simulink model "deltino"  (R2021b)
settings: Solver=VariableStepAuto  StartTime=0.0  StopTime=inf  FixedStep=0.0001  RelTol=1e-3
values from neighbouring files (symbols this model uses):
  alpha1 = 0    [compute_deltino_dyn_parallel.m]
  alpha2 = 2/3*pi    (= 2.09439510239)    [compute_deltino_dyn_parallel.m]
  alpha3 = 4/3*pi    (= 4.18879020479)    [compute_deltino_dyn_parallel.m]
  H = 0.05    [main.m]
  J_T = [J_1', J_2', J_3', J_4']    [main.m]
  K_d = 10    [main.m]
  K_el = 10000    [main.m]
  K_i = 1    [main.m]
  K_p = 200    [main.m]
  K_v = 10    [main.m]
  mu = 0.8    [main.m]
  ni_0 = zeros(18,1)    [main.m]
  offset1 = [l1/2; l2/2; -h/2]    [compute_deltino_dyn_parallel.m]    (also in main.m = [+l1/2; +l2/2; -h/2])
  offset2 = [l1/2; -l2/2; -h/2]    [compute_deltino_dyn_parallel.m]    (also in main.m = [+l1/2; -l2/2; -h/2])
  offset3 = [-l1/2; -l2/2; -h/2]    [compute_deltino_dyn_parallel.m]    (also in main.m)
  offset4 = [-l1/2; l2/2; -h/2]    [compute_deltino_dyn_parallel.m]    (also in main.m = [-l1/2; +l2/2; -h/2])
  p_leg1_0 = forward_kin(theta_leg1_0)    [main.m]
  p_leg2_0 = forward_kin(theta_leg2_0)    [main.m]
  p_leg3_0 = forward_kin(theta_leg3_0)    [main.m]
  p_leg4_0 = forward_kin(theta_leg4_0)    [main.m]
  points_ccw = [+0.1,  0.00 ... (first row only)    [main.m]
  points_cw = [-0.1,  0.00 ... (first row only)    [main.m]
  q_0 = [base_0; ypr_0; theta_leg1_0; ee_leg1_0; theta_leg2_0; ee_leg2_0;        theta_leg3_0; ee_leg3_0; theta_leg4_0; ee_leg4_0;]    [main.m]
  ratio = 2    [main.m]
  steps = 4+2*ratio    (= 8)    [main.m]
  theta_leg1_0 = [pi/6; pi/6; pi/6]    [main.m]
  theta_leg2_0 = [pi/6; pi/6; pi/6]    [main.m]
  theta_leg3_0 = [pi/6; pi/6; pi/6]    [main.m]
  theta_leg4_0 = [pi/6; pi/6; pi/6]    [main.m]
  ts = T/steps    (= 0.1875)    [main.m]
  ts2 = 3*ts    (= 0.5625)    [main.m]
  vel = 0.2    [main.m]
undefined symbols (not defined in the file or in its folder): l1, l_A, l_B, R, radius0, radius1, radius2, theta, WPs
libraries: simulink x14, dspsigops x12
(part 6 of 10)

== matlab function deltino/DELTINO DYNAMICS /compute_M ==
  data: q input; M output
function M = M(q)
%#codegen

%    This function was generated by the Symbolic Math Toolbox version 9.0.
%    03-May-2022 23:36:54
phi = q(4); zeta = q(5); psi = q(6);
th11 = q(7); th12 = q(8); th13 = q(9);
th21 = q(13); th22 = q(14); th23 = q(15);
th31 = q(19); th32 = q(20); th33 = q(21);
th41 = q(25); th42 = q(26); th43 = q(27);


t2 = cos(phi);
t3 = cos(psi);
t4 = cos(th11);
t5 = cos(th12);
t6 = cos(th13);
t7 = cos(th21);
t8 = cos(th22);
t9 = cos(th23);
t10 = cos(th31);
t11 = cos(th32);
t12 = cos(th33);
t13 = cos(th41);
t14 = cos(th42);
t15 = cos(th43);
t16 = cos(zeta);
t17 = sin(phi);
t18 = sin(psi);
t19 = sin(th11);
t20 = sin(th12);
t21 = sin(th13);
t22 = sin(th21);
t23 = sin(th22);
t24 = sin(th23);
t25 = sin(th31);
t26 = sin(th32);
t27 = sin(th33);
t28 = sin(th41);
t29 = sin(th42);
t30 = sin(th43);
t31 = sin(zeta);
t32 = psi.*2.0;
t33 = th11.*2.0;
t34 = th12.*2.0;
t35 = th13.*2.0;
t36 = th21.*2.0;
t37 = th22.*2.0;
t38 = th23.*2.0;
t39 = th31.*2.0;
t40 = th32.*2.0;
t41 = th33.*2.0;
t42 = th41.*2.0;
t43 = th42.*2.0;
t44 = th43.*2.0;
t94 = sqrt(3.0);
t95 = psi./2.0;
t96 = th12./2.0;
t97 = th13./2.0;
t98 = th22./2.0;
t99 = th23./2.0;
t100 = th32./2.0;
t101 = th33./2.0;
t102 = th42./2.0;
t103 = th43./2.0;
t45 = cos(t32);
t46 = t3.^2;
t47 = cos(t34);
t48 = cos(t35);
t49 = cos(t37);
t50 = cos(t38);
t51 = cos(t40);
t52 = cos(t41);
t53 = cos(t43);
t54 = cos(t44);
t55 = t4.^2;
t56 = t5.^2;
t57 = t6.^2;
t58 = t7.^2;
t59 = t8.^2;
t60 = t9.^2;
t61 = t10.^2;
t62 = t11.^2;
t63 = t12.^2;
t64 = t13.^2;
t65 = t14.^2;
t66 = t15.^2;
t67 = t16.^2;
t68 = sin(t32);
t69 = sin(t33);
t70 = sin(t34);
t71 = sin(t35);
t72 = sin(t36);
t73 = sin(t37);
t74 = sin(t38);
t75 = sin(t39);
t76 = sin(t40);
t77 = sin(t41);
t78 = sin(t42);
t79 = sin(t43);
t80 = sin(t44);
t81 = t2.*t3;
t82 = t2.*t18;
t83 = t3.*t17;
t84 = t5.*t31;
t85 = t6.*t31;
t86 = t8.*t31;
t87 = t9.*t31;
t88 = t11.*t31;
t89 = t12.*t31;
t90 = t14.*t31;
t91 = t15.*t31;
t92 = t17.*t18;
t93 = t18.*1.6e+1;
t104 = t4.*t31.*2.0;
t105 = t7.*t31.*2.0;
t106 = t10.*t31.*2.0;
t107 = t13.*t31.*2.0;
t108 = t18.*t19.*2.0;
t109 = t18.*t20.*2.0;
t110 = t18.*t21.*2.0;
t111 = t18.*t22.*2.0;
t112 = t18.*t23.*2.0;
t113 = t18.*t24.*2.0;
t114 = t18.*t25.*2.0;
t115 = t18.*t26.*2.0;
t116 = t18.*t27.*2.0;
t117 = t18.*t28.*2.0;
t118 = t18.*t29.*2.0;
t119 = t18.*t30.*2.0;
t120 = cos(t95);
t121 = cos(t96);
t122 = cos(t97);
t123 = cos(t98);
t124 = cos(t99);
t125 = cos(t100);
t126 = cos(t101);
t127 = cos(t102);
t128 = cos(t103);
t129 = t16./2.0;
t130 = sin(t95);
t131 = sin(t96);
t132 = sin(t97);
t133 = sin(t98);
t134 = sin(t99);
t135 = sin(t100);
t136 = sin(t101);
t137 = sin(t102);
t138 = sin(t103);
t139 = t31./2.0;
t142 = t3.*t16.*1.6e+1;
t152 = t4.*(3.0./2.0e+1);
t153 = t5.*(3.0./2.0e+1);
t154 = t6.*(3.0./2.0e+1);
t155 = t7.*(3.0./2.0e+1);
t156 = t8.*(3.0./2.0e+1);
t157 = t9.*(3.0./2.0e+1);
t158 = t10.*(3.0./2.0e+1);
t159 = t11.*(3.0./2.0e+1);
t160 = t12.*(3.0./2.0e+1);
t161 = t13.*(3.0./2.0e+1);
t162 = t14.*(3.0./2.0e+1);
t163 = t15.*(3.0./2.0e+1);
t164 = t16.*(6.0./2.5e+1);
t169 = t3.*(4.0./3.75e+2);
t180 = t3.*t16.*t19.*2.0;
t181 = t3.*t16.*t20.*2.0;
t182 = t3.*t16.*t21.*2.0;
t183 = t3.*t16.*t22.*2.0;
t184 = t3.*t16.*t23.*2.0;
t185 = t3.*t16.*t24.*2.0;
t186 = t3.*t16.*t25.*2.0;
t187 = t3.*t16.*t26.*2.0;
t188 = t3.*t16.*t27.*2.0;
t189 = t3.*t16.*t28.*2.0;
t190 = t3.*t16.*t29.*2.0;
t191 = t3.*t16.*t30.*2.0;
t195 = t2.*t16.*(7.0./2.0e+1);
t196 = t4.*t16.*(3.0./5.0e+1);
t197 = t7.*t16.*(3.0./5.0e+1);
t198 = t10.*t16.*(3.0./5.0e+1);
t199 = t13.*t16.*(3.0./5.0e+1);
t202 = t16.*t17.*(7.0./2.0e+1);
t204 = t19.*t31.*(3.0./5.0e+1);
t205 = t22.*t31.*(3.0./5.0e+1);
t206 = t25.*t31.*(3.0./5.0e+1);
t207 = t28.*t31.*(3.0./5.0e+1);
t209 = t3.*t4.*(3.0./1.0e+2);
t210 = t3.*t7.*(3.0./1.0e+2);
t211 = t3.*t10.*(3.0./2.5e+2);
t212 = t3.*t13.*(3.0./2.5e+2);
t222 = t3.*t19.*(3.0./5.0e+2);
t223 = t4.*t18.*(3.0./5.0e+2);
t224 = t3.*t22.*(3.0./5.0e+2);
t225 = t7.*t18.*(3.0./5.0e+2);
t226 = t3.*t25.*(3.0./5.0e+2);
t227 = t10.*t18.*(3.0./5.0e+2);
t228 = t3.*t28.*(3.0./5.0e+2);
t229 = t13.*t18.*(3.0./5.0e+2);
t231 = t3.*t31.*(1.2e+1./2.5e+1);
t232 = t16.*t18.*(2.0./3.75e+2);
t233 = t16.*t18.*(4.0./3.75e+2);
t235 = t18.*t19.*(3.0./1.0e+2);
t236 = t18.*t22.*(3.0./1.0e+2);
t237 = t18.*t25.*(3.0./2.5e+2);
t238 = t18.*t28.*(3.0./2.5e+2);
t239 = t19.*t31.*(3.0./2.5e+2);
t240 = t20.*t31.*(3.0./2.5e+2);
t241 = t21.*t31.*(3.0./2.5e+2);
t242 = t22.*t31.*(3.0./2.5e+2);
t243 = t23.*t31.*(3.0./2.5e+2);
t244 = t24.*t31.*(3.0./2.5e+2);
t245 = t25.*t31.*(3.0./2.5e+2);
t246 = t26.*t31.*(3.0./2.5e+2);
t247 = t27.*t31.*(3.0./2.5e+2);
t248 = t28.*t31.*(3.0./2.5e+2);
t249 = t29.*t31.*(3.0./2.5e+2);
t250 = t30.*t31.*(3.0./2.5e+2);
t251 = t4.*(2.1e+1./1.0e+3);
t252 = t5.*(2.1e+1./1.0e+3);
t253 = t6.*(2.1e+1./1.0e+3);
t254 = t7.*(2.1e+1./1.0e+3);
t255 = t8.*(2.1e+1./1.0e+3);
t256 = t9.*(2.1e+1./1.0e+3);
t257 = t10.*(2.1e+1./1.0e+3);
t258 = t11.*(2.1e+1./1.0e+3);
t259 = t12.*(2.1e+1./1.0e+3);
t260 = t13.*(2.1e+1./1.0e+3);
t261 = t14.*(2.1e+1./1.0e+3);
t262 = t15.*(2.1e+1./1.0e+3);
t263 = t3.*t5.*t94;
t264 = t3.*t6.*t94;
t265 = t3.*t8.*t94;
t266 = t3.*t9.*t94;
t267 = t3.*t11.*t94;
t268 = t3.*t12.*t94;
t269 = t3.*t14.*t94;
t270 = t3.*t15.*t94;
t273 = t16.*t17.*t19.*(3.0./5.0e+1);
t274 = t16.*t17.*t22.*(3.0./5.0e+1);
t275 = t16.*t17.*t25.*(3.0./5.0e+1);
t276 = t16.*t17.*t28.*(3.0./5.0e+1);
t278 = t3.*t20.*t31.*(3.0./5.0e+1);
t279 = t3.*t21.*t31.*(3.0./5.0e+1);
t281 = t3.*t23.*t31.*(3.0./5.0e+1);
t282 = t3.*t24.*t31.*(3.0./5.0e+1);
t284 = t3.*t26.*t31.*(3.0./5.0e+1);
t285 = t3.*t27.*t31.*(3.0./5.0e+1);
t287 = t3.*t29.*t31.*(3.0./5.0e+1);
t288 = t3.*t30.*t31.*(3.0./5.0e+1);
t298 = t5.*t18.*(3.0./1.0e+3);
t299 = t6.*t18.*(3.0./1.0e+3);
t300 = t8.*t18.*(3.0./1.0e+3);
t301 = t9.*t18.*(3.0./1.0e+3);
t302 = t11.*t18.*(3.0./1.0e+3);
t303 = t12.*t18.*(3.0./1.0e+3);
t304 = t14.*t18.*(3.0./1.0e+3);
t305 = t15.*t18.*(3.0./1.0e+3);
t307 = (t16.*t18)./1.2e+3;
t330 = t94.*(2.0./3.75e+2);
t332 = t3.*t5.*t16.*(3.0./5.0e+1);
t333 = t3.*t6.*t16.*(3.0./5.0e+1);
t335 = t3.*t8.*t16.*(3.0./5.0e+1);
t336 = t3.*t9.*t16.*(3.0./5.0e+1);
t338 = t3.*t11.*t16.*(3.0./5.0e+1);
t339 = t3.*t12.*t16.*(3.0./5.0e+1);
t341 = t3.*t14.*t16.*(3.0./5.0e+1);
t342 = t3.*t15.*t16.*(3.0./5.0e+1);
t344 = t2.*t16.*t19.*(3.0./5.0e+1);
t345 = t2.*t16.*t22.*(3.0./5.0e+1);
t346 = t2.*t16.*t25.*(3.0./5.0e+1);
t347 = t2.*t16.*t28.*(3.0./5.0e+1);
t357 = t16.*t18.*t19.*(3.0./5.0e+2);
t359 = t16.*t18.*t22.*(3.0./5.0e+2);
t361 = t16.*t18.*t25.*(3.0./5.0e+2);
t363 = t16.*t18.*t28.*(3.0./5.0e+2);
t368 = t3.*t5.*1.05e-2;
t369 = t3.*t6.*1.05e-2;
t370 = t3.*t8.*1.05e-2;
t371 = t3.*t9.*1.05e-2;
t372 = t3.*t11.*1.05e-2;
t373 = t3.*t12.*1.05e-2;
t374 = t3.*t14.*1.05e-2;
t375 = t3.*t15.*1.05e-2;
t382 = t16.*t19.*(2.1e+1./1.0e+3);
t384 = t16.*t20.*(2.1e+1./1.0e+3);
t386 = t16.*t21.*(2.1e+1./1.0e+3);
t388 = t16.*t22.*(2.1e+1./1.0e+3);
t390 = t16.*t23.*(2.1e+1./1.0e+3);
t392 = t16.*t24.*(2.1e+1./1.0e+3);
t394 = t16.*t25.*(2.1e+1./1.0e+3);
t396 = t16.*t26.*(2.1e+1./1.0e+3);
t398 = t16.*t27.*(2.1e+1./1.0e+3);
t400 = t16.*t28.*(2.1e+1./1.0e+3);
t402 = t16.*t29.*(2.1e+1./1.0e+3);
t404 = t16.*t30.*(2.1e+1./1.0e+3);
t413 = t18.*t19.*(2.1e+1./1.0e+3);
t414 = t18.*t22.*(2.1e+1./1.0e+3);
t415 = t18.*t25.*(2.1e+1./1.0e+3);
t416 = t18.*t28.*(2.1e+1./1.0e+3);
t417 = t18.*t20.*1.65e-2;
t418 = t18.*t21.*1.65e-2;
t419 = t18.*t23.*1.65e-2;
t420 = t18.*t24.*1.65e-2;
t421 = t18.*t26.*2.55e-2;
t422 = t18.*t27.*2.55e-2;
t423 = t18.*t29.*2.55e-2;
t424 = t18.*t30.*2.55e-2;
t425 = t5.*t16.*t18.*t94;
t426 = t6.*t16.*t18.*t94;
t427 = t8.*t16.*t18.*t94;
t428 = t9.*t16.*t18.*t94;
t429 = t11.*t16.*t18.*t94;
t430 = t12.*t16.*t18.*t94;
t431 = t14.*t16.*t18.*t94;
t432 = t15.*t16.*t18.*t94;
t474 = t3.*t4.*t16.*(-3.0./5.0e+1);
t477 = t3.*t7.*t16.*(-3.0./5.0e+1);
t480 = t3.*t10.*t16.*(-3.0./5.0e+1);
t483 = t3.*t13.*t16.*(-3.0./5.0e+1);
t486 = t3.*t4.*t16.*(3.0./5.0e+2);
t487 = t3.*t7.*t16.*(3.0./5.0e+2);
t488 = t3.*t10.*t16.*(3.0./5.0e+2);
t489 = t3.*t13.*t16.*(3.0./5.0e+2);
t495 = t3.*t16.*t19.*(3.0./1.0e+2);
t496 = t4.*t16.*t18.*(3.0./1.0e+2);
t497 = t3.*t16.*t22.*(3.0./1.0e+2);
t498 = t7.*t16.*t18.*(3.0./1.0e+2);
t499 = t3.*t16.*t25.*(3.0./2.5e+2);
t500 = t10.*t16.*t18.*(3.0./2.5e+2);
t501 = t3.*t16.*t28.*(3.0./2.5e+2);
t502 = t13.*t16.*t18.*(3.0./2.5e+2);
t504 = t16.*t18.*t20.*(3.0./1.0e+3);
t506 = t16.*t18.*t21.*(3.0./1.0e+3);
t508 = t16.*t18.*t23.*(3.0./1.0e+3);
t510 = t16.*t18.*t24.*(3.0./1.0e+3);
t512 = t16.*t18.*t26.*(3.0./1.0e+3);
t514 = t16.*t18.*t27.*(3.0./1.0e+3);
t516 = t16.*t18.*t29.*(3.0./1.0e+3);
t518 = t16.*t18.*t30.*(3.0./1.0e+3);
t519 = t3.*t4.*(-2.1e+1./1.0e+3);
t520 = t3.*t13.*(-2.1e+1./1.0e+3);
t525 = t18.*t25.*t31.*(-3.0./2.5e+2);
t526 = t18.*t28.*t31.*(-3.0./2.5e+2);
t530 = t7.*t31.*(-2.1e+1./1.0e+3);
t533 = t10.*t31.*(-2.1e+1./1.0e+3);
t562 = t3.*t5.*t16.*(3.0./1.0e+3);
t563 = t3.*t6.*t16.*(3.0./1.0e+3);
t564 = t3.*t8.*t16.*(3.0./1.0e+3);
t565 = t3.*t9.*t16.*(3.0./1.0e+3);
t566 = t3.*t11.*t16.*(3.0./1.0e+3);
t567 = t3.*t12.*t16.*(3.0./1.0e+3);
t568 = t3.*t14.*t16.*(3.0./1.0e+3);
t569 = t3.*t15.*t16.*(3.0./1.0e+3);
t599 = t31.*8.229e-1;
t604 = t16.*t18.*t94.*(-1.0./2.0);
t605 = t18.*t31.*t94.*(-1.0./2.0);
t606 = t20.*t94.*(3.0./1.0e+3);
t607 = t21.*t94.*(3.0./1.0e+3);
t608 = t23.*t94.*(3.0./1.0e+3);
t609 = t24.*t94.*(3.0./1.0e+3);
t610 = t26.*t94.*(3.0./1.0e+3);
t611 = t27.*t94.*(3.0./1.0e+3);
t612 = t29.*t94.*(3.0./1.0e+3);
t613 = t30.*t94.*(3.0./1.0e+3);
t614 = t31.*t94.*(-2.0./3.75e+2);
t615 = (t31.*t94)./1.2e+3;
t617 = t3.*t5.*t16.*t20.*(2.0./3.75e+2);
t618 = t3.*t6.*t16.*t21.*(2.0./3.75e+2);
t620 = t3.*t8.*t16.*t23.*(2.0./3.75e+2);
t621 = t3.*t9.*t16.*t24.*(2.0./3.75e+2);
t623 = t3.*t11.*t16.*t26.*(2.0./3.75e+2);
t624 = t3.*t12.*t16.*t27.*(2.0./3.75e+2);
t626 = t3.*t14.*t16.*t29.*(2.0./3.75e+2);
t627 = t3.*t15.*t16.*t30.*(2.0./3.75e+2);
t628 = t3.*t16.*t18.*t19.*(3.0./2.5e+2);
t629 = t3.*t16.*t18.*t20.*(3.0./2.5e+2);
t630 = t3.*t16.*t18.*t21.*(3.0./2.5e+2);
t631 = t3.*t16.*t18.*t22.*(3.0./2.5e+2);
t632 = t3.*t16.*t18.*t23.*(3.0./2.5e+2);
t633 = t3.*t16.*t18.*t24.*(3.0./2.5e+2);
t635 = t3.*t16.*t18.*t26.*(3.0./2.5e+2);
t636 = t3.*t16.*t18.*t27.*(3.0./2.5e+2);
t638 = t3.*t16.*t18.*t29.*(3.0./2.5e+2);
t639 = t3.*t16.*t18.*t30.*(3.0./2.5e+2);
t648 = t4.*t18.*t19.*t31.*(4.0./3.75e+2);
t651 = t7.*t18.*t22.*t31.*(4.0./3.75e+2);
t654 = t10.*t18.*t25.*t31.*(4.0./3.75e+2);
t657 = t13.*t18.*t28.*t31.*(4.0./3.75e+2);
t673 = t3.*t16.*t20.*1.05e-2;
t674 = t5.*t16.*t18.*1.05e-2;
t676 = t3.*t16.*t21.*1.05e-2;
t677 = t6.*t16.*t18.*1.05e-2;
t679 = t3.*t16.*t23.*1.05e-2;
t680 = t8.*t16.*t18.*1.05e-2;
t682 = t3.*t16.*t24.*1.05e-2;
t683 = t9.*t16.*t18.*1.05e-2;
t684 = t3.*t16.*t20.*1.65e-2;
t685 = t5.*t16.*t18.*1.65e-2;
t686 = t3.*t16.*t21.*1.65e-2;
t687 = t6.*t16.*t18.*1.65e-2;
t689 = t3.*t16.*t26.*1.05e-2;
t690 = t11.*t16.*t18.*1.05e-2;
t692 = t3.*t16.*t27.*1.05e-2;
t693 = t12.*t16.*t18.*1.05e-2;
t694 = t3.*t16.*t23.*1.65e-2;
t695 = t8.*t16.*t18.*1.65e-2;
t696 = t3.*t16.*t24.*1.65e-2;
t697 = t9.*t16.*t18.*1.65e-2;
t699 = t3.*t16.*t29.*1.05e-2;
t700 = t14.*t16.*t18.*1.05e-2;
t702 = t3.*t16.*t30.*1.05e-2;
t703 = t15.*t16.*t18.*1.05e-2;
t704 = t3.*t16.*t26.*2.55e-2;
t705 = t11.*t16.*t18.*2.55e-2;
t706 = t3.*t16.*t27.*2.55e-2;
t707 = t12.*t16.*t18.*2.55e-2;
t708 = t3.*t16.*t29.*2.55e-2;
t709 = t14.*t16.*t18.*2.55e-2;
t710 = t3.*t16.*t30.*2.55e-2;
t711 = t15.*t16.*t18.*2.55e-2;
t712 = t18.*t26.*t31.*(-2.55e-2);
t713 = t18.*t27.*t31.*(-2.55e-2);
t714 = t18.*t29.*t31.*(-2.55e-2);
t715 = t18.*t30.*t31.*(-2.55e-2);
t739 = t5.*t94.*4.5e-3;
t740 = t6.*t94.*4.5e-3;
t741 = t8.*t94.*4.5e-3;
t742 = t9.*t94.*4.5e-3;
t743 = t11.*t94.*4.5e-3;
t744 = t12.*t94.*4.5e-3;
t745 = t14.*t94.*4.5e-3;
t746 = t15.*t94.*4.5e-3;
t767 = t4.*t16.*t18.*(-2.1e+1./1.0e+3);
t769 = t3.*t16.*t22.*(-2.1e+1./1.0e+3);
t771 = t3.*t16.*t25.*(-2.1e+1./1.0e+3);
t772 = t13.*t16.*t18.*(-2.1e+1./1.0e+3);
t815 = t5.*t16.*t94.*(3.0./1.0e+3);
t816 = t6.*t16.*t94.*(3.0./1.0e+3);
t817 = t8.*t16.*t94.*(3.0./1.0e+3);
t818 = t9.*t16.*t94.*(3.0./1.0e+3);
t819 = t11.*t16.*t94.*(3.0./1.0e+3);
t820 = t12.*t16.*t94.*(3.0./1.0e+3);
t821 = t14.*t16.*t94.*(3.0./1.0e+3);
t822 = t15.*t16.*t94.*(3.0./1.0e+3);
t835 = t3.*t5.*t16.*t18.*1.35e-2;
t836 = t3.*t6.*t16.*t18.*1.35e-2;
t837 = t3.*t8.*t16.*t18.*1.35e-2;
t838 = t3.*t9.*t16.*t18.*1.35e-2;
t839 = t3.*t11.*t16.*t18.*1.35e-2;
t840 = t3.*t12.*t16.*t18.*1.35e-2;
t841 = t3.*t14.*t16.*t18.*1.35e-2;
t842 = t3.*t15.*t16.*t18.*1.35e-2;
t843 = t3.*t16.*t18.*5.21125e-1;
t901 = t16.*t20.*t94.*4.5e-3;
t903 = t16.*t21.*t94.*4.5e-3;
t905 = t16.*t23.*t94.*4.5e-3;
t907 = t16.*t24.*t94.*4.5e-3;
t909 = t16.*t26.*t94.*4.5e-3;
t911 = t16.*t27.*t94.*4.5e-3;
t913 = t16.*t29.*t94.*4.5e-3;
t915 = t16.*t30.*t94.*4.5e-3;
t916 = t21.*t31.*t94.*(-3.0./1.0e+3);
t917 = t24.*t31.*t94.*(-3.0./1.0e+3);
t918 = t27.*t31.*t94.*(-3.0./1.0e+3);
t919 = t30.*t31.*t94.*(-3.0./1.0e+3);
t943 = t5.*t16.*t20.*t94.*(-2.0./3.75e+2);
t944 = t8.*t16.*t23.*t94.*(-2.0./3.75e+2);
t945 = t11.*t16.*t26.*t94.*(-2.0./3.75e+2);
t946 = t14.*t16.*t29.*t94.*(-2.0./3.75e+2);
t1014 = t3.*t16.*t20.*t94.*(-1.05e-2);
t1015 = t3.*t16.*t23.*t94.*(-1.05e-2);
t1016 = t3.*t16.*t27.*t94.*(-1.05e-2);
t1017 = t3.*t16.*t30.*t94.*(-1.05e-2);
t140 = t31.*t82;
t141 = t31.*t83;
t143 = t31.*t92;
t144 = -t84;
t145 = -t85;
t146 = -t86;
t147 = -t87;
t148 = -t88;
t149 = -t89;
t150 = -t90;
t151 = -t91;
t165 = t31.*t81;
t166 = t2.*t129;
t167 = t17.*t129;
t168 = t18.*t129;
t170 = -t164;
t171 = t120.^2;
t172 = t121.^2;
t173 = t122.^2;
t174 = t123.^2;
t175 = t124.^2;
t176 = t125.^2;
t177 = t126.^2;
t178 = t127.^2;
t179 = t128.^2;
t194 = t81.*(7.0./2.0e+1);
t200 = t82./1.0e+1;
t201 = t83.*(7.0./2.0e+1);
t203 = t92./1.0e+1;
t208 = t81.*(1.2e+1./2.5e+1);
t213 = -t195;
t214 = -t196;
t215 = -t197;
t216 = -t198;
t217 = -t199;
t220 = t82.*(1.2e+1./2.5e+1);
t221 = t83.*(1.2e+1./2.5e+1);
t230 = -t202;
M = ft_1({t10,t1014,t1015,t1016,t1017,t104,t105,t106,t107,t108,t109,t11,t110,t111,t112,t113,t114,t115,t116,t117,t118,t119,t12,t120,t121,t122,t123,t124,t125,t126,t127,t128,t129,t13,t130,t131,t132,t133,t134,t135,t136,t137,t138,t139,t14,t140,t141,t142,t143,t144,t145,t146,t147,t148,t149,t15,t150,t151,t152,t153,t154,t155,t156,t157,t158,t159,t16,t160,t161,t162,t163,t165,t166,t167,t168,t169,t17,t170,t171,t172,t173,t174,t175,t176,t177,t178,t179,t18,t180,t181,t182,t183,t184,t185,t186,t187,t188,t189,t19,t190,t191,t194,t195,t196,t197,t198,t199,t2,t20,t200,t201,t202,t203,t204,t205,t206,t207,t208,t209,t21,t210,t211,t212,t213,t214,t215,t216,t217,t22,t220,t221,t222,t223,t224,t225,t226,t227,t228,t229,t23,t230,t231,t232,t233,t235,t236,t237,t238,t239,t24,t240,t241,t242,t243,t244,t245,t246,t247,t248,t249,t25,t250,t251,t252,t253,t254,t255,t256,t257,t258,t259,t26,t260,t261,t262,t263,t264,t265,t266,t267,t268,t269,t27,t270,t273,t274,t275,t276,t278,t279,t28,t281,t282,t284,t285,t287,t288,t29,t298,t299,t3,t30,t300,t301,t302,t303,t304,t305,t307,t31,t330,t332,t333,t335,t336,t338,t339,t341,t342,t344,t345,t346,t347,t357,t359,t361,t363,t368,t369,t370,t371,t372,t373,t374,t375,t382,t384,t386,t388,t390,t392,t394,t396,t398,t4,t400,t402,t404,t413,t414,t415,t416,t417,t418,t419,t420,t421,t422,t423,t424,t425,t426,t427,t428,t429,t430,t431,t432,t45,t46,t47,t474,t477,t48,t480,t483,t486,t487,t488,t489,t49,t495,t496,t497,t498,t499,t5,t50,t500,t501,t502,t504,t506,t508,t51,t510,t512,t514,t516,t518,t519,t52,t520,t525,t526,t53,t530,t533,t54,t55,t56,t562,t563,t564,t565,t566,t567,t568,t569,t57,t58,t59,t599,t6,t60,t604,t605,t606,t607,t608,t609,t61,t610,t611,t612,t613,t614,t615,t617,t618,t62,t620,t621,t623,t624,t626,t627,t628,t629,t63,t630,t631,t632,t633,t635,t636,t638,t639,t64,t648,t65,t651,t654,t657,t66,t67,t673,t674,t676,t677,t679,t68,t680,t682,t683,t684,t685,t686,t687,t689,t69,t690,t692,t693,t694,t695,t696,t697,t699,t7,t70,t700,t702,t703,t704,t705,t706,t707,t708,t709,t71,t710,t711,t712,t713,t714,t715,t72,t73,t739,t74,t740,t741,t742,t743,t744,t745,t746,t75,t76,t767,t769,t77,t771,t772,t78,t79,t8,t80,t81,t815,t816,t817,t818,t819,t82,t820,t821,t822,t83,t835,t836,t837,t838,t839,t84,t840,t841,t842,t843,t85,t86,t87,t88,t89,t9,t90,t901,t903,t905,t907,t909,t91,t911,t913,t915,t916,t917,t918,t919,t92,t93,t94,t943,t944,t945,t946});
end
function M = ft_1(ct)
t10 = ct{1};
t1014 = ct{2};
t1015 = ct{3};
t1016 = ct{4};
t1017 = ct{5};
t104 = ct{6};
t105 = ct{7};
t106 = ct{8};
t107 = ct{9};
t108 = ct{10};
t109 = ct{11};
t11 = ct{12};
t110 = ct{13};
t111 = ct{14};
t112 = ct{15};
t113 = ct{16};
t114 = ct{17};
t115 = ct{18};
t116 = ct{19};
t117 = ct{20};
t118 = ct{21};
t119 = ct{22};
t12 = ct{23};
t120 = ct{24};
t121 = ct{25};
t122 = ct{26};
t123 = ct{27};
t124 = ct{28};
t125 = ct{29};
t126 = ct{30};
t127 = ct{31};
t128 = ct{32};
t129 = ct{33};
t13 = ct{34};
t130 = ct{35};
t131 = ct{36};
t132 = ct{37};
t133 = ct{38};
t134 = ct{39};
t135 = ct{40};
t136 = ct{41};
t137 = ct{42};
t138 = ct{43};
t139 = ct{44};
t14 = ct{45};
t140 = ct{46};
t141 = ct{47};
t142 = ct{48};
t143 = ct{49};
t144 = ct{50};
t145 = ct{51};
t146 = ct{52};
t147 = ct{53};
t148 = ct{54};
t149 = ct{55};
t15 = ct{56};
t150 = ct{57};
t151 = ct{58};
t152 = ct{59};
t153 = ct{60};
t154 = ct{61};
t155 = ct{62};
t156 = ct{63};
t157 = ct{64};
t158 = ct{65};
t159 = ct{66};
t16 = ct{67};
t160 = ct{68};
t161 = ct{69};
t162 = ct{70};
t163 = ct{71};
t165 = ct{72};
t166 = ct{73};
t167 = ct{74};
t168 = ct{75};
t169 = ct{76};
t17 = ct{77};
t170 = ct{78};
t171 = ct{79};
t172 = ct{80};
t173 = ct{81};
t174 = ct{82};
t175 = ct{83};
t176 = ct{84};
t177 = ct{85};
t178 = ct{86};
t179 = ct{87};
t18 = ct{88};
t180 = ct{89};
t181 = ct{90};
t182 = ct{91};
t183 = ct{92};
t184 = ct{93};
t185 = ct{94};
t186 = ct{95};
t187 = ct{96};
t188 = ct{97};
t189 = ct{98};
t19 = ct{99};
t190 = ct{100};
t191 = ct{101};
t194 = ct{102};
t195 = ct{103};
t196 = ct{104};
t197 = ct{105};
t198 = ct{106};
t199 = ct{107};
t2 = ct{108};
t20 = ct{109};
t200 = ct{110};
t201 = ct{111};
t202 = ct{112};
t203 = ct{113};
t204 = ct{114};
t205 = ct{115};
t206 = ct{116};
t207 = ct{117};
t208 = ct{118};
t209 = ct{119};
t21 = ct{120};
t210 = ct{121};
t211 = ct{122};
t212 = ct{123};
t213 = ct{124};
t214 = ct{125};
t215 = ct{126};
t216 = ct{127};
t217 = ct{128};
t22 = ct{129};
t220 = ct{130};
t221 = ct{131};
t222 = ct{132};
t223 = ct{133};
t224 = ct{134};
t225 = ct{135};
t226 = ct{136};
t227 = ct{137};
t228 = ct{138};
t229 = ct{139};
t23 = ct{140};
t230 = ct{141};
t231 = ct{142};
t232 = ct{143};
t233 = ct{144};
t235 = ct{145};
t236 = ct{146};
t237 = ct{147};
t238 = ct{148};
t239 = ct{149};
t24 = ct{150};
t240 = ct{151};
t241 = ct{152};
t242 = ct{153};
t243 = ct{154};
t244 = ct{155};
t245 = ct{156};
t246 = ct{157};
t247 = ct{158};
t248 = ct{159};
t249 = ct{160};
t25 = ct{161};
t250 = ct{162};
t251 = ct{163};
t252 = ct{164};
t253 = ct{165};
t254 = ct{166};
t255 = ct{167};
t256 = ct{168};
t257 = ct{169};
t258 = ct{170};
t259 = ct{171};
t26 = ct{172};
t260 = ct{173};
t261 = ct{174};
t262 = ct{175};
t263 = ct{176};
t264 = ct{177};
t265 = ct{178};
t266 = ct{179};
t267 = ct{180};
t268 = ct{181};
t269 = ct{182};
t27 = ct{183};
t270 = ct{184};
t273 = ct{185};
t274 = ct{186};
t275 = ct{187};
t276 = ct{188};
t278 = ct{189};
t279 = ct{190};
t28 = ct{191};
t281 = ct{192};
t282 = ct{193};
t284 = ct{194};
t285 = ct{195};
t287 = ct{196};
t288 = ct{197};
t29 = ct{198};
t298 = ct{199};
t299 = ct{200};
t3 = ct{201};
t30 = ct{202};
t300 = ct{203};
t301 = ct{204};
t302 = ct{205};
t303 = ct{206};
t304 = ct{207};
t305 = ct{208};
t307 = ct{209};
t31 = ct{210};
t330 = ct{211};
t332 = ct{212};
t333 = ct{213};
t335 = ct{214};
t336 = ct{215};
t338 = ct{216};
t339 = ct{217};
t341 = ct{218};
t342 = ct{219};
t344 = ct{220};
t345 = ct{221};
t346 = ct{222};
t347 = ct{223};
t357 = ct{224};
t359 = ct{225};
t361 = ct{226};
t363 = ct{227};
t368 = ct{228};
t369 = ct{229};
t370 = ct{230};
t371 = ct{231};
t372 = ct{232};
t373 = ct{233};
t374 = ct{234};
t375 = ct{235};
t382 = ct{236};
t384 = ct{237};
t386 = ct{238};
t388 = ct{239};
t390 = ct{240};
t392 = ct{241};
t394 = ct{242};
t396 = ct{243};
t398 = ct{244};
t4 = ct{245};
t400 = ct{246};
t402 = ct{247};
t404 = ct{248};
t413 = ct{249};
t414 = ct{250};
t415 = ct{251};
t416 = ct{252};
t417 = ct{253};
t418 = ct{254};
t419 = ct{255};
t420 = ct{256};
t421 = ct{257};
t422 = ct{258};
t423 = ct{259};
t424 = ct{260};
t425 = ct{261};
t426 = ct{262};
t427 = ct{263};
t428 = ct{264};
t429 = ct{265};
t430 = ct{266};
t431 = ct{267};
t432 = ct{268};
t45 = ct{269};
t46 = ct{270};
t47 = ct{271};
t474 = ct{272};
t477 = ct{273};
t48 = ct{274};
t480 = ct{275};
t483 = ct{276};
t486 = ct{277};
t487 = ct{278};
t488 = ct{279};
t489 = ct{280};
t49 = ct{281};
t495 = ct{282};
t496 = ct{283};
t497 = ct{284};
t498 = ct{285};
t499 = ct{286};
t5 = ct{287};
t50 = ct{288};
t500 = ct{289};
t501 = ct{290};
t502 = ct{291};
t504 = ct{292};
t506 = ct{293};
t508 = ct{294};
t51 = ct{295};
t510 = ct{296};
t512 = ct{297};
t514 = ct{298};
t516 = ct{299};
t518 = ct{300};
t519 = ct{301};
t52 = ct{302};
t520 = ct{303};
t525 = ct{304};
t526 = ct{305};
t53 = ct{306};
t530 = ct{307};
t533 = ct{308};
t54 = ct{309};
t55 = ct{310};
t56 = ct{311};
t562 = ct{312};
t563 = ct{313};
t564 = ct{314};
t565 = ct{315};
t566 = ct{316};
t567 = ct{317};
t568 = ct{318};
t569 = ct{319};
t57 = ct{320};
t58 = ct{321};
t59 = ct{322};
t599 = ct{323};
t6 = ct{324};
t60 = ct{325};
t604 = ct{326};
t605 = ct{327};
t606 = ct{328};
t607 = ct{329};
t608 = ct{330};
t609 = ct{331};
t61 = ct{332};
t610 = ct{333};
t611 = ct{334};
t612 = ct{335};
t613 = ct{336};
t614 = ct{337};
t615 = ct{338};
t617 = ct{339};
t618 = ct{340};
t62 = ct{341};
t620 = ct{342};
t621 = ct{343};
t623 = ct{344};
t624 = ct{345};
t626 = ct{346};
t627 = ct{347};
t628 = ct{348};
t629 = ct{349};
t63 = ct{350};
t630 = ct{351};
t631 = ct{352};
t632 = ct{353};
t633 = ct{354};
t635 = ct{355};
t636 = ct{356};
t638 = ct{357};
t639 = ct{358};
t64 = ct{359};
t648 = ct{360};
t65 = ct{361};
t651 = ct{362};
t654 = ct{363};
t657 = ct{364};
t66 = ct{365};
t67 = ct{366};
t673 = ct{367};
t674 = ct{368};
t676 = ct{369};
t677 = ct{370};
t679 = ct{371};
t68 = ct{372};
t680 = ct{373};
t682 = ct{374};
t683 = ct{375};
t684 = ct{376};
t685 = ct{377};
t686 = ct{378};
t687 = ct{379};
t689 = ct{380};
t69 = ct{381};
t690 = ct{382};
t692 = ct{383};
t693 = ct{384};
t694 = ct{385};
t695 = ct{386};
t696 = ct{387};
t697 = ct{388};
t699 = ct{389};
t7 = ct{390};
t70 = ct{391};
t700 = ct{392};
t702 = ct{393};
t703 = ct{394};
t704 = ct{395};
t705 = ct{396};
t706 = ct{397};
t707 = ct{398};
t708 = ct{399};
t709 = ct{400};
t71 = ct{401};
t710 = ct{402};
t711 = ct{403};
t712 = ct{404};
t713 = ct{405};
t714 = ct{406};
t715 = ct{407};
t72 = ct{408};
t73 = ct{409};
t739 = ct{410};
t74 = ct{411};
t740 = ct{412};
t741 = ct{413};
t742 = ct{414};
t743 = ct{415};
t744 = ct{416};
t745 = ct{417};
t746 = ct{418};
t75 = ct{419};
t76 = ct{420};
t767 = ct{421};
t769 = ct{422};
t77 = ct{423};
t771 = ct{424};
t772 = ct{425};
t78 = ct{426};
t79 = ct{427};
t8 = ct{428};
t80 = ct{429};
t81 = ct{430};
t815 = ct{431};
t816 = ct{432};
t817 = ct{433};
t818 = ct{434};
t819 = ct{435};
t82 = ct{436};
t820 = ct{437};
t821 = ct{438};
t822 = ct{439};
t83 = ct{440};
t835 = ct{441};
t836 = ct{442};
t837 = ct{443};
t838 = ct{444};
t839 = ct{445};
t84 = ct{446};
t840 = ct{447};
t841 = ct{448};
t842 = ct{449};
t843 = ct{450};
t85 = ct{451};
t86 = ct{452};
t87 = ct{453};
t88 = ct{454};
t89 = ct{455};
t9 = ct{456};
t90 = ct{457};
t901 = ct{458};
t903 = ct{459};
t905 = ct{460};
t907 = ct{461};
t909 = ct{462};
t91 = ct{463};
t911 = ct{464};
t913 = ct{465};
t915 = ct{466};
t916 = ct{467};
t917 = ct{468};
t918 = ct{469};
t919 = ct{470};
t92 = ct{471};
t93 = ct{472};
t94 = ct{473};
t943 = ct{474};
t944 = ct{475};
t945 = ct{476};
t946 = ct{477};
t234 = t92.*(1.2e+1./2.5e+1);
t277 = t3.*t204;
t280 = t3.*t205;
t283 = t3.*t206;
t286 = t3.*t207;
t289 = -t211;
t290 = -t212;
t294 = -t223;
t295 = -t225;
t296 = -t227;
t297 = -t229;
t306 = -t232;
t309 = -t235;
t310 = -t236;
t311 = -t239;
t312 = -t240;
t313 = -t241;
t314 = -t242;
t315 = -t243;
t316 = -t244;
t317 = -t245;
t318 = -t246;
t319 = -t247;
t320 = -t248;
t321 = -t249;
t322 = -t250;
t323 = -t251;
t324 = -t252;
t325 = -t253;
t326 = -t260;
t327 = -t261;
t328 = -t262;
t329 = t94.*t139;
t331 = t3.*t196;
t334 = t3.*t197;
t337 = t3.*t198;
t340 = t3.*t199;
t352 = -t273;
t353 = -t274;
t354 = -t275;
t355 = -t276;
t356 = t31.*t223;
t358 = t31.*t225;
t360 = t31.*t227;
t362 = t31.*t229;
t364 = t3.*t251;
t365 = t3.*t254;
t366 = t3.*t257;
t367 = t3.*t260;
t377 = t31.*t235;
t378 = t31.*t236;
t379 = t31.*t237;
t380 = t31.*t238;
t381 = t31.*t251;
t383 = t84.*(2.1e+1./1.0e+3);
t385 = t85.*(2.1e+1./1.0e+3);
t387 = t31.*t254;
t389 = t86.*(2.1e+1./1.0e+3);
t391 = t87.*(2.1e+1./1.0e+3);
t393 = t31.*t257;
t395 = t88.*(2.1e+1./1.0e+3);
t397 = t89.*(2.1e+1./1.0e+3);
t399 = t31.*t260;
t401 = t90.*(2.1e+1./1.0e+3);
t403 = t91.*(2.1e+1./1.0e+3);
t405 = t84.*1.35e-2;
t406 = t85.*1.35e-2;
t407 = t86.*1.35e-2;
t408 = t87.*1.35e-2;
t409 = t88.*1.35e-2;
t410 = t89.*1.35e-2;
t411 = t90.*1.35e-2;
t412 = t91.*1.35e-2;
t433 = -t264;
t434 = -t266;
t435 = -t268;
t436 = -t270;
t437 = (t31.*t56)./3.75e+2;
t438 = (t31.*t57)./3.75e+2;
t439 = t31.*t55.*(4.0./3.75e+2);
t440 = (t31.*t59)./3.75e+2;
t441 = (t31.*t60)./3.75e+2;
t442 = t31.*t58.*(4.0./3.75e+2);
t443 = (t31.*t62)./3.75e+2;
t444 = (t31.*t63)./3.75e+2;
t445 = t31.*t61.*(4.0./3.75e+2);
t446 = (t31.*t65)./3.75e+2;
t447 = (t31.*t66)./3.75e+2;
t448 = t31.*t64.*(4.0./3.75e+2);
t449 = t18.*t69.*(2.0./3.75e+2);
t450 = (t18.*t70)./3.75e+2;
t451 = (t18.*t71)./3.75e+2;
t452 = t18.*t72.*(2.0./3.75e+2);
t453 = (t18.*t73)./3.75e+2;
t454 = (t18.*t74)./3.75e+2;
t455 = t18.*t75.*(2.0./3.75e+2);
t456 = (t18.*t76)./3.75e+2;
t457 = (t18.*t77)./3.75e+2;
t458 = t18.*t78.*(2.0./3.75e+2);
t459 = (t18.*t79)./3.75e+2;
t460 = (t18.*t80)./3.75e+2;
t461 = t152+3.0./2.0e+1;
t462 = t153+3.0./2.0e+1;
t463 = t154+3.0./2.0e+1;
t464 = t155+3.0./2.0e+1;
t465 = t156+3.0./2.0e+1;
t466 = t157+3.0./2.0e+1;
t467 = t158+3.0./2.0e+1;
t468 = t159+3.0./2.0e+1;
t469 = t160+3.0./2.0e+1;
t470 = t161+3.0./2.0e+1;
t471 = t162+3.0./2.0e+1;
t472 = t163+3.0./2.0e+1;
t473 = -t330;
t475 = -t332;
t476 = -t333;
t478 = -t335;
t479 = -t336;
t481 = -t338;
t482 = -t339;
t484 = -t341;
t485 = -t342;
t491 = -t344;
t492 = -t345;
t493 = -t346;
t494 = -t347;
t503 = t18.*t84.*(3.0./1.0e+3);
t505 = t18.*t85.*(3.0./1.0e+3);
t507 = t18.*t86.*(3.0./1.0e+3);
t509 = t18.*t87.*(3.0./1.0e+3);
t511 = t18.*t88.*(3.0./1.0e+3);
t513 = t18.*t89.*(3.0./1.0e+3);
t515 = t18.*t90.*(3.0./1.0e+3);
t517 = t18.*t91.*(3.0./1.0e+3);
t521 = -t370;
t522 = -t371;
t523 = -t372;
t524 = -t373;
t527 = -t382;
t528 = -t384;
t529 = -t386;
t536 = -t400;
t537 = -t402;
t538 = -t404;
t547 = -t413;
t548 = -t416;
t549 = -t417;
t550 = -t418;
t551 = -t419;
t552 = -t420;
t561 = t31.*t330;
t571 = -t499;
t572 = -t500;
t573 = -t501;
t574 = -t502;
t576 = -t504;
t578 = -t506;
t580 = -t508;
t582 = -t510;
t584 = -t512;
t586 = -t514;
t588 = -t516;
t590 = -t518;
t591 = t31.*t417;
t592 = t31.*t418;
t593 = t31.*t419;
t594 = t31.*t420;
t595 = t31.*t421;
t596 = t31.*t422;
t597 = t31.*t423;
t598 = t31.*t424;
t600 = -t425;
t601 = -t427;
t602 = -t429;
t603 = -t431;
t616 = t4.*t16.*t19.*t169;
t619 = t7.*t16.*t22.*t169;
t622 = t10.*t16.*t25.*t169;
t625 = t13.*t16.*t28.*t169;
t634 = t3.*t16.*t237;
t637 = t3.*t16.*t238;
t640 = -t562;
t641 = -t563;
t642 = -t564;
t643 = -t565;
t644 = -t566;
t645 = -t567;
t646 = -t568;
t647 = -t569;
t649 = t18.*t20.*t84.*(2.0./3.75e+2);
t650 = t18.*t21.*t85.*(2.0./3.75e+2);
t652 = t18.*t23.*t86.*(2.0./3.75e+2);
t653 = t18.*t24.*t87.*(2.0./3.75e+2);
t655 = t18.*t26.*t88.*(2.0./3.75e+2);
t656 = t18.*t27.*t89.*(2.0./3.75e+2);
t658 = t18.*t29.*t90.*(2.0./3.75e+2);
t659 = t18.*t30.*t91.*(2.0./3.75e+2);
t661 = t3.*t382;
t662 = t16.*t18.*t251;
t664 = t3.*t388;
t665 = t16.*t18.*t254;
t667 = t3.*t394;
t668 = t16.*t18.*t257;
t670 = t3.*t400;
t671 = t16.*t18.*t260;
t672 = t3.*t84.*1.05e-2;
t675 = t3.*t85.*1.05e-2;
t678 = t3.*t86.*1.05e-2;
t681 = t3.*t87.*1.05e-2;
t688 = t3.*t88.*1.05e-2;
t691 = t3.*t89.*1.05e-2;
t698 = t3.*t90.*1.05e-2;
t701 = t3.*t91.*1.05e-2;
t716 = -t599;
t717 = t16.*t19.*t46.*(2.1e+1./5.0e+2);
t718 = t16.*t20.*t46.*(2.1e+1./5.0e+2);
t719 = t16.*t21.*t46.*(2.1e+1./5.0e+2);
t720 = t16.*t22.*t46.*(2.1e+1./5.0e+2);
t721 = t16.*t23.*t46.*(2.1e+1./5.0e+2);
t722 = t16.*t24.*t46.*(2.1e+1./5.0e+2);
t723 = t16.*t25.*t46.*(2.1e+1./5.0e+2);
t724 = t16.*t26.*t46.*(2.1e+1./5.0e+2);
t725 = t16.*t27.*t46.*(2.1e+1./5.0e+2);
t726 = t16.*t28.*t46.*(2.1e+1./5.0e+2);
t727 = t16.*t29.*t46.*(2.1e+1./5.0e+2);
t728 = t16.*t30.*t46.*(2.1e+1./5.0e+2);
t729 = t267.*(3.0./2.0e+2);
t730 = t268.*(3.0./2.0e+2);
t731 = t269.*(3.0./2.0e+2);
t732 = t270.*(3.0./2.0e+2);
t733 = t263.*(3.0./5.0e+2);
t734 = t264.*(3.0./5.0e+2);
t735 = t265.*(3.0./5.0e+2);
t736 = t266.*(3.0./5.0e+2);
t747 = -t606;
t748 = -t608;
t749 = -t610;
t750 = -t612;
t751 = -t617;
t752 = -t618;
t753 = -t620;
t754 = -t621;
t755 = -t623;
t756 = -t624;
t757 = -t626;
t758 = -t627;
t768 = t3.*t530;
t770 = t3.*t533;
t774 = -t673;
t776 = -t676;
t777 = -t680;
t778 = -t683;
t779 = -t690;
t780 = -t693;
t782 = -t699;
t784 = -t702;
t785 = -t704;
t786 = -t705;
t787 = -t706;
t788 = -t707;
t789 = -t708;
t790 = -t709;
t791 = -t710;
t792 = -t711;
t793 = t16.*t18.*t55.*t169;
t794 = t3.*t16.*t18.*t56.*(7.0./3.75e+2);
t795 = t3.*t16.*t18.*t57.*(7.0./3.75e+2);
t796 = t16.*t18.*t58.*t169;
t797 = t3.*t16.*t18.*t59.*(7.0./3.75e+2);
t798 = t3.*t16.*t18.*t60.*(7.0./3.75e+2);
t799 = t16.*t18.*t61.*t169;
t800 = t3.*t16.*t18.*t62.*(7.0./3.75e+2);
t801 = t3.*t16.*t18.*t63.*(7.0./3.75e+2);
t802 = t16.*t18.*t64.*t169;
t803 = t3.*t16.*t18.*t65.*(7.0./3.75e+2);
t804 = t3.*t16.*t18.*t66.*(7.0./3.75e+2);
t823 = t31.*t606;
t824 = t31.*t607;
t825 = t31.*t608;
t826 = t31.*t609;
t827 = t31.*t610;
t828 = t31.*t611;
t829 = t31.*t612;
t830 = t31.*t613;
t831 = -t739;
t832 = -t741;
t833 = -t743;
t834 = -t745;
t852 = t3.*t16.*t18.*t55.*(-4.0./3.75e+2);
t855 = t3.*t16.*t18.*t58.*(-4.0./3.75e+2);
t858 = t3.*t16.*t18.*t61.*(-4.0./3.75e+2);
t861 = t3.*t16.*t18.*t64.*(-4.0./3.75e+2);
t864 = t3.*t88.*t94.*(3.0./2.0e+2);
t865 = t429.*(3.0./2.0e+2);
t866 = t3.*t89.*t94.*(3.0./2.0e+2);
t867 = t430.*(3.0./2.0e+2);
t868 = t3.*t90.*t94.*(3.0./2.0e+2);
t869 = t431.*(3.0./2.0e+2);
t870 = t3.*t91.*t94.*(3.0./2.0e+2);
t871 = t432.*(3.0./2.0e+2);
t872 = t3.*t84.*t94.*(3.0./5.0e+2);
t873 = t425.*(3.0./5.0e+2);
t874 = t3.*t85.*t94.*(3.0./5.0e+2);
t875 = t426.*(3.0./5.0e+2);
t876 = t3.*t86.*t94.*(3.0./5.0e+2);
t877 = t427.*(3.0./5.0e+2);
t878 = t3.*t87.*t94.*(3.0./5.0e+2);
t879 = t428.*(3.0./5.0e+2);
t880 = t5.*t16.*t20.*t330;
t881 = t6.*t16.*t21.*t330;
t882 = t8.*t16.*t23.*t330;
t883 = t9.*t16.*t24.*t330;
t884 = t11.*t16.*t26.*t330;
t885 = t12.*t16.*t27.*t330;
t886 = t14.*t16.*t29.*t330;
t887 = t15.*t16.*t30.*t330;
t888 = -t815;
t889 = -t817;
t890 = -t819;
t891 = -t821;
t900 = t84.*t94.*4.5e-3;
t902 = t85.*t94.*4.5e-3;
t904 = t86.*t94.*4.5e-3;
t906 = t87.*t94.*4.5e-3;
t908 = t88.*t94.*4.5e-3;
t910 = t89.*t94.*4.5e-3;
t912 = t90.*t94.*4.5e-3;
t914 = t91.*t94.*4.5e-3;
t920 = -t835;
t921 = -t836;
t922 = -t837;
t923 = -t838;
t924 = -t839;
t925 = -t840;
t926 = -t841;
t927 = -t842;
t930 = -t843;
t947 = t84.*t94.*(-2.1e+1./1.0e+3);
t948 = t87.*t94.*(-2.1e+1./1.0e+3);
t949 = t89.*t94.*(-2.1e+1./1.0e+3);
t950 = t90.*t94.*(-2.1e+1./1.0e+3);
t951 = -t901;
t953 = -t905;
t955 = -t909;
t957 = -t913;
t959 = (t3.*t47.*t94)./7.5e+2;
t960 = (t3.*t48.*t94)./7.5e+2;
t961 = (t3.*t49.*t94)./7.5e+2;
t962 = (t3.*t50.*t94)./7.5e+2;
t963 = (t3.*t51.*t94)./7.5e+2;
t964 = (t3.*t52.*t94)./7.5e+2;
t965 = (t3.*t53.*t94)./7.5e+2;
t966 = (t3.*t54.*t94)./7.5e+2;
t967 = t121.*t131.*(3.0./5.0e+2);
t968 = t122.*t132.*(3.0./5.0e+2);
t969 = t123.*t133.*(3.0./5.0e+2);
t970 = t124.*t134.*(3.0./5.0e+2);
t971 = t125.*t135.*(3.0./5.0e+2);
t972 = t126.*t136.*(3.0./5.0e+2);
t973 = t127.*t137.*(3.0./5.0e+2);
t974 = t128.*t138.*(3.0./5.0e+2);
t976 = t94.*t673;
t977 = t94.*t676;
t978 = t94.*t679;
t979 = t94.*t682;
t980 = t94.*t689;
t981 = t94.*t692;
t982 = t94.*t699;
t983 = t94.*t702;
t984 = t5.*t16.*t46.*t94.*(3.0./5.0e+2);
t985 = t6.*t16.*t46.*t94.*(3.0./5.0e+2);
t986 = t8.*t16.*t46.*t94.*(3.0./5.0e+2);
t987 = t9.*t16.*t46.*t94.*(3.0./5.0e+2);
t988 = t11.*t16.*t46.*t94.*(3.0./5.0e+2);
t989 = t12.*t16.*t46.*t94.*(3.0./5.0e+2);
t990 = t14.*t16.*t46.*t94.*(3.0./5.0e+2);
t991 = t15.*t16.*t46.*t94.*(3.0./5.0e+2);
t993 = (t16.*t18.*t56.*t94)./3.75e+2;
t995 = (t16.*t18.*t57.*t94)./3.75e+2;
t997 = (t16.*t18.*t59.*t94)./3.75e+2;
t999 = (t16.*t18.*t60.*t94)./3.75e+2;
t1001 = (t16.*t18.*t62.*t94)./3.75e+2;
t1003 = (t16.*t18.*t63.*t94)./3.75e+2;
t1005 = (t16.*t18.*t65.*t94)./3.75e+2;
t1007 = (t16.*t18.*t66.*t94)./3.75e+2;
t1042 = t3.*t31.*t56.*t94.*(-1.0./3.75e+2);
t1044 = t3.*t31.*t59.*t94.*(-1.0./3.75e+2);
t1046 = t3.*t31.*t62.*t94.*(-1.0./3.75e+2);
t1048 = t3.*t31.*t65.*t94.*(-1.0./3.75e+2);
t1074 = t3.*t16.*t18.*t94.*t252;
t1075 = t3.*t16.*t18.*t94.*t253;
t1076 = t3.*t16.*t18.*t94.*t255;
t1077 = t3.*t16.*t18.*t94.*t256;
t1078 = t3.*t16.*t18.*t94.*t258;
t1079 = t3.*t16.*t18.*t94.*t259;
t1080 = t3.*t16.*t18.*t94.*t261;
t1081 = t3.*t16.*t18.*t94.*t262;
t1082 = t129+t605;
t1083 = t139+t604;
t1084 = t5.*t16.*t20.*t46.*t94.*(4.0./3.75e+2);
t1085 = t6.*t16.*t21.*t46.*t94.*(4.0./3.75e+2);
t1086 = t8.*t16.*t23.*t46.*t94.*(4.0./3.75e+2);
t1087 = t9.*t16.*t24.*t46.*t94.*(4.0./3.75e+2);
t1088 = t11.*t16.*t26.*t46.*t94.*(4.0./3.75e+2);
t1089 = t12.*t16.*t27.*t46.*t94.*(4.0./3.75e+2);
t1090 = t14.*t16.*t29.*t46.*t94.*(4.0./3.75e+2);
t1091 = t15.*t16.*t30.*t46.*t94.*(4.0./3.75e+2);
t1108 = t16.*t20.*t46.*t94.*(9.0./1.0e+3);
t1109 = t16.*t21.*t46.*t94.*(9.0./1.0e+3);
t1110 = t16.*t23.*t46.*t94.*(9.0./1.0e+3);
t1111 = t16.*t24.*t46.*t94.*(9.0./1.0e+3);
t1112 = t16.*t26.*t46.*t94.*(9.0./1.0e+3);
t1113 = t16.*t27.*t46.*t94.*(9.0./1.0e+3);
t1114 = t16.*t29.*t46.*t94.*(9.0./1.0e+3);
t1115 = t16.*t30.*t46.*t94.*(9.0./1.0e+3);
t1128 = t16.*t18.*t263.*(-2.1e+1./1.0e+3);
t1129 = t16.*t18.*t266.*(-2.1e+1./1.0e+3);
t1130 = t16.*t18.*t268.*(-2.1e+1./1.0e+3);
t1131 = t16.*t18.*t269.*(-2.1e+1./1.0e+3);
t1133 = t204+t474;
t1134 = t205+t477;
t1135 = t206+t480;
t1136 = t207+t483;
t1252 = t120.*t121.*t130.*t131.*(2.1e+1./5.0e+2);
t1253 = t120.*t122.*t130.*t132.*(2.1e+1./5.0e+2);
t1254 = t120.*t123.*t130.*t133.*(2.1e+1./5.0e+2);
t1255 = t120.*t124.*t130.*t134.*(2.1e+1./5.0e+2);
t1256 = t120.*t125.*t130.*t135.*(2.1e+1./5.0e+2);
t1257 = t120.*t126.*t130.*t136.*(2.1e+1./5.0e+2);
t1258 = t120.*t127.*t130.*t137.*(2.1e+1./5.0e+2);
t1259 = t120.*t128.*t130.*t138.*(2.1e+1./5.0e+2);
t1312 = t94.*t120.*t122.*t130.*t132.*(-2.1e+1./5.0e+2);
t1313 = t94.*t120.*t124.*t130.*t134.*(-2.1e+1./5.0e+2);
t1314 = t94.*t120.*t125.*t130.*t135.*(-2.1e+1./5.0e+2);
t1315 = t94.*t120.*t127.*t130.*t137.*(-2.1e+1./5.0e+2);
t1336 = t169+t210+t224+t414;
t1368 = t256+t330+t609+t742;
t1369 = t259+t330+t611+t744;
t1398 = t233+t359+t498+t530+t769;
t192 = -t140;
t193 = -t141;
t218 = -t200;
t219 = -t201;
t271 = t141./1.0e+1;
t272 = t140.*(7.0./2.0e+1);
t291 = t143.*(7.0./2.0e+1);
t292 = -t220;
t293 = -t221;
t308 = -t234;
t343 = t165./1.0e+1;
t350 = t140.*(1.2e+1./2.5e+1);
t351 = t141.*(1.2e+1./2.5e+1);
t376 = t143.*(1.2e+1./2.5e+1);
t490 = t165.*(1.2e+1./2.5e+1);
t531 = -t389;
t532 = -t391;
t534 = -t395;
t535 = -t397;
t539 = -t405;
t540 = -t406;
t541 = -t407;
t542 = -t408;
t543 = -t409;
t544 = -t410;
t545 = -t411;
t546 = -t412;
t553 = t81+t143;
t554 = t92+t165;
t555 = t94.*t168;
t556 = -t449;
t557 = -t452;
t558 = -t455;
t559 = -t458;
t560 = t18.*t329;
t575 = -t503;
t577 = -t505;
t579 = -t507;
t581 = -t509;
t583 = -t511;
t585 = -t513;
t587 = -t515;
t589 = -t517;
t660 = t31.*t364;
t663 = t31.*t365;
t666 = t31.*t366;
t669 = t31.*t367;
t759 = -t649;
t760 = -t650;
t761 = -t652;
t762 = -t653;
t763 = -t655;
t764 = -t656;
t765 = -t658;
t766 = -t659;
t773 = -t672;
t775 = -t675;
t781 = -t698;
t783 = -t701;
t805 = -t720;
t806 = -t721;
M = ft_2({t10,t1001,t1003,t1005,t1007,t1014,t1015,t1016,t1017,t104,t1042,t1044,t1046,t1048,t105,t106,t107,t1075,t1076,t1078,t108,t1081,t1082,t1083,t1084,t1085,t1086,t1087,t1088,t1089,t109,t1090,t1091,t11,t110,t1108,t1109,t111,t1110,t1111,t1112,t1113,t1114,t1115,t112,t1128,t1129,t113,t1130,t1131,t1133,t1134,t1135,t1136,t114,t115,t116,t117,t118,t119,t12,t121,t122,t123,t124,t125,t1252,t1253,t1254,t1255,t1256,t1257,t1258,t1259,t126,t127,t128,t129,t13,t131,t1312,t1313,t1314,t1315,t132,t133,t1336,t134,t135,t136,t1368,t1369,t137,t138,t139,t1398,t14,t142,t144,t145,t146,t147,t148,t149,t15,t150,t151,t16,t166,t167,t168,t169,t17,t170,t171,t172,t173,t174,t175,t176,t177,t178,t179,t18,t180,t181,t182,t183,t184,t185,t186,t187,t188,t189,t19,t190,t191,t192,t193,t194,t195,t2,t20,t200,t201,t202,t203,t208,t209,t21,t213,t214,t215,t216,t217,t218,t219,t22,t222,t226,t228,t23,t230,t231,t233,t237,t238,t24,t25,t252,t254,t255,t256,t257,t258,t259,t26,t261,t263,t265,t267,t269,t27,t271,t272,t277,t278,t279,t28,t280,t281,t282,t283,t284,t285,t286,t287,t288,t289,t29,t290,t291,t292,t293,t294,t295,t296,t297,t298,t299,t3,t30,t300,t301,t302,t303,t304,t305,t306,t307,t308,t309,t31,t310,t311,t312,t313,t314,t315,t316,t317,t318,t319,t320,t321,t322,t323,t324,t325,t326,t327,t328,t329,t330,t343,t350,t351,t352,t353,t354,t355,t356,t357,t358,t360,t361,t362,t363,t365,t366,t368,t369,t374,t375,t376,t377,t378,t381,t383,t385,t388,t389,t390,t391,t392,t394,t395,t396,t397,t398,t399,t4,t401,t403,t415,t421,t422,t423,t424,t426,t428,t430,t432,t433,t434,t435,t436,t437,t438,t439,t440,t441,t442,t443,t444,t445,t446,t447,t448,t45,t450,t451,t453,t454,t456,t457,t459,t46,t460,t461,t462,t463,t464,t465,t466,t467,t468,t469,t470,t471,t472,t473,t475,t476,t478,t479,t481,t482,t484,t485,t486,t487,t488,t489,t490,t491,t492,t493,t494,t495,t496,t497,t5,t519,t520,t521,t522,t523,t524,t525,t526,t527,t528,t529,t531,t532,t533,t534,t535,t536,t537,t538,t539,t540,t541,t542,t543,t544,t545,t546,t547,t548,t549,t55,t550,t551,t552,t553,t554,t555,t556,t557,t558,t559,t56,t560,t561,t57,t571,t572,t573,t574,t575,t576,t577,t578,t579,t58,t580,t581,t582,t583,t584,t585,t586,t587,t588,t589,t59,t590,t591,t592,t593,t594,t6,t60,t600,t601,t602,t603,t607,t61,t613,t614,t615,t616,t619,t62,t622,t625,t628,t629,t63,t630,t631,t632,t633,t634,t635,t636,t637,t638,t639,t64,t640,t641,t642,t643,t644,t645,t646,t647,t648,t65,t651,t654,t657,t66,t660,t661,t665,t668,t669,t67,t670,t674,t677,t678,t679,t68,t681,t682,t684,t685,t686,t687,t688,t689,t691,t692,t694,t695,t696,t697,t7,t700,t703,t712,t713,t714,t715,t716,t717,t718,t719,t722,t723,t724,t725,t726,t727,t728,t729,t730,t731,t732,t733,t734,t735,t736,t740,t746,t747,t748,t749,t750,t751,t752,t753,t754,t755,t756,t757,t758,t759,t760,t761,t762,t763,t764,t765,t766,t767,t768,t770,t771,t772,t773,t774,t775,t776,t777,t778,t779,t780,t781,t782,t783,t784,t785,t786,t787,t788,t789,t790,t791,t792,t794,t795,t797,t798,t8,t800,t801,t803,t804,t805,t806,t816,t818,t82,t820,t822,t823,t825,t827,t829,t83,t831,t832,t833,t834,t852,t855,t858,t861,t864,t865,t866,t867,t868,t869,t870,t871,t872,t873,t874,t875,t876,t877,t878,t879,t881,t883,t885,t887,t888,t889,t890,t891,t9,t900,t902,t903,t904,t906,t907,t908,t910,t911,t912,t914,t915,t916,t917,t918,t919,t920,t921,t922,t923,t924,t925,t926,t927,t93,t930,t94,t943,t944,t945,t946,t947,t948,t949,t950,t951,t953,t955,t957,t959,t960,t961,t962,t963,t964,t965,t966,t967,t968,t969,t970,t971,t972,t973,t974,t977,t979,t980,t982,t984,t985,t986,t987,t988,t989,t990,t991,t993,t995,t997,t999});
end
function M = ft_2(ct)
t10 = ct{1};
t1001 = ct{2};
t1003 = ct{3};
t1005 = ct{4};
t1007 = ct{5};
t1014 = ct{6};
t1015 = ct{7};
t1016 = ct{8};
t1017 = ct{9};
t104 = ct{10};
t1042 = ct{11};
t1044 = ct{12};
t1046 = ct{13};
t1048 = ct{14};
t105 = ct{15};
t106 = ct{16};
t107 = ct{17};
t1075 = ct{18};
t1076 = ct{19};
t1078 = ct{20};
t108 = ct{21};
t1081 = ct{22};
t1082 = ct{23};
t1083 = ct{24};
t1084 = ct{25};
t1085 = ct{26};
t1086 = ct{27};
t1087 = ct{28};
t1088 = ct{29};
t1089 = ct{30};
t109 = ct{31};
t1090 = ct{32};
t1091 = ct{33};
t11 = ct{34};
t110 = ct{35};
t1108 = ct{36};
t1109 = ct{37};
t111 = ct{38};
t1110 = ct{39};
t1111 = ct{40};
t1112 = ct{41};
t1113 = ct{42};
t1114 = ct{43};
t1115 = ct{44};
t112 = ct{45};
t1128 = ct{46};
t1129 = ct{47};
t113 = ct{48};
t1130 = ct{49};
t1131 = ct{50};
t1133 = ct{51};
t1134 = ct{52};
t1135 = ct{53};
t1136 = ct{54};
t114 = ct{55};
t115 = ct{56};
t116 = ct{57};
t117 = ct{58};
t118 = ct{59};
t119 = ct{60};
t12 = ct{61};
t121 = ct{62};
t122 = ct{63};
t123 = ct{64};
t124 = ct{65};
t125 = ct{66};
t1252 = ct{67};
t1253 = ct{68};
t1254 = ct{69};
t1255 = ct{70};
t1256 = ct{71};
t1257 = ct{72};
t1258 = ct{73};
t1259 = ct{74};
t126 = ct{75};
t127 = ct{76};
t128 = ct{77};
t129 = ct{78};
t13 = ct{79};
t131 = ct{80};
t1312 = ct{81};
t1313 = ct{82};
t1314 = ct{83};
t1315 = ct{84};
t132 = ct{85};
t133 = ct{86};
t1336 = ct{87};
t134 = ct{88};
t135 = ct{89};
t136 = ct{90};
t1368 = ct{91};
t1369 = ct{92};
t137 = ct{93};
t138 = ct{94};
t139 = ct{95};
t1398 = ct{96};
t14 = ct{97};
t142 = ct{98};
t144 = ct{99};
t145 = ct{100};
t146 = ct{101};
t147 = ct{102};
t148 = ct{103};
t149 = ct{104};
t15 = ct{105};
t150 = ct{106};
t151 = ct{107};
t16 = ct{108};
t166 = ct{109};
t167 = ct{110};
t168 = ct{111};
t169 = ct{112};
t17 = ct{113};
t170 = ct{114};
t171 = ct{115};
t172 = ct{116};
t173 = ct{117};
t174 = ct{118};
t175 = ct{119};
t176 = ct{120};
t177 = ct{121};
t178 = ct{122};
t179 = ct{123};
t18 = ct{124};
t180 = ct{125};
t181 = ct{126};
t182 = ct{127};
t183 = ct{128};
t184 = ct{129};
t185 = ct{130};
t186 = ct{131};
t187 = ct{132};
t188 = ct{133};
t189 = ct{134};
t19 = ct{135};
t190 = ct{136};
t191 = ct{137};
t192 = ct{138};
t193 = ct{139};
t194 = ct{140};
t195 = ct{141};
t2 = ct{142};
t20 = ct{143};
t200 = ct{144};
t201 = ct{145};
t202 = ct{146};
t203 = ct{147};
t208 = ct{148};
t209 = ct{149};
t21 = ct{150};
t213 = ct{151};
t214 = ct{152};
t215 = ct{153};
t216 = ct{154};
t217 = ct{155};
t218 = ct{156};
t219 = ct{157};
t22 = ct{158};
t222 = ct{159};
t226 = ct{160};
t228 = ct{161};
t23 = ct{162};
t230 = ct{163};
t231 = ct{164};
t233 = ct{165};
t237 = ct{166};
t238 = ct{167};
t24 = ct{168};
t25 = ct{169};
t252 = ct{170};
t254 = ct{171};
t255 = ct{172};
t256 = ct{173};
t257 = ct{174};
t258 = ct{175};
t259 = ct{176};
t26 = ct{177};
t261 = ct{178};
t263 = ct{179};
t265 = ct{180};
t267 = ct{181};
t269 = ct{182};
t27 = ct{183};
t271 = ct{184};
t272 = ct{185};
t277 = ct{186};
t278 = ct{187};
t279 = ct{188};
t28 = ct{189};
t280 = ct{190};
t281 = ct{191};
t282 = ct{192};
t283 = ct{193};
t284 = ct{194};
t285 = ct{195};
t286 = ct{196};
t287 = ct{197};
t288 = ct{198};
t289 = ct{199};
t29 = ct{200};
t290 = ct{201};
t291 = ct{202};
t292 = ct{203};
t293 = ct{204};
t294 = ct{205};
t295 = ct{206};
t296 = ct{207};
t297 = ct{208};
t298 = ct{209};
t299 = ct{210};
t3 = ct{211};
t30 = ct{212};
t300 = ct{213};
t301 = ct{214};
t302 = ct{215};
t303 = ct{216};
t304 = ct{217};
t305 = ct{218};
t306 = ct{219};
t307 = ct{220};
t308 = ct{221};
t309 = ct{222};
t31 = ct{223};
t310 = ct{224};
t311 = ct{225};
t312 = ct{226};
t313 = ct{227};
t314 = ct{228};
t315 = ct{229};
t316 = ct{230};
t317 = ct{231};
t318 = ct{232};
t319 = ct{233};
t320 = ct{234};
t321 = ct{235};
t322 = ct{236};
t323 = ct{237};
t324 = ct{238};
t325 = ct{239};
t326 = ct{240};
t327 = ct{241};
t328 = ct{242};
t329 = ct{243};
t330 = ct{244};
t343 = ct{245};
t350 = ct{246};
t351 = ct{247};
t352 = ct{248};
t353 = ct{249};
t354 = ct{250};
t355 = ct{251};
t356 = ct{252};
t357 = ct{253};
t358 = ct{254};
t360 = ct{255};
t361 = ct{256};
t362 = ct{257};
t363 = ct{258};
t365 = ct{259};
t366 = ct{260};
t368 = ct{261};
t369 = ct{262};
t374 = ct{263};
t375 = ct{264};
t376 = ct{265};
t377 = ct{266};
t378 = ct{267};
t381 = ct{268};
t383 = ct{269};
t385 = ct{270};
t388 = ct{271};
t389 = ct{272};
t390 = ct{273};
t391 = ct{274};
t392 = ct{275};
t394 = ct{276};
t395 = ct{277};
t396 = ct{278};
t397 = ct{279};
t398 = ct{280};
t399 = ct{281};
t4 = ct{282};
t401 = ct{283};
t403 = ct{284};
t415 = ct{285};
t421 = ct{286};
t422 = ct{287};
t423 = ct{288};
t424 = ct{289};
t426 = ct{290};
t428 = ct{291};
t430 = ct{292};
t432 = ct{293};
t433 = ct{294};
t434 = ct{295};
t435 = ct{296};
t436 = ct{297};
t437 = ct{298};
t438 = ct{299};
t439 = ct{300};
t440 = ct{301};
t441 = ct{302};
t442 = ct{303};
t443 = ct{304};
t444 = ct{305};
t445 = ct{306};
t446 = ct{307};
t447 = ct{308};
t448 = ct{309};
t45 = ct{310};
t450 = ct{311};
t451 = ct{312};
t453 = ct{313};
t454 = ct{314};
t456 = ct{315};
t457 = ct{316};
t459 = ct{317};
t46 = ct{318};
t460 = ct{319};
t461 = ct{320};
t462 = ct{321};
t463 = ct{322};
t464 = ct{323};
t465 = ct{324};
t466 = ct{325};
t467 = ct{326};
t468 = ct{327};
t469 = ct{328};
t470 = ct{329};
t471 = ct{330};
t472 = ct{331};
t473 = ct{332};
t475 = ct{333};
t476 = ct{334};
t478 = ct{335};
t479 = ct{336};
t481 = ct{337};
t482 = ct{338};
t484 = ct{339};
t485 = ct{340};
t486 = ct{341};
t487 = ct{342};
t488 = ct{343};
t489 = ct{344};
t490 = ct{345};
t491 = ct{346};
t492 = ct{347};
t493 = ct{348};
t494 = ct{349};
t495 = ct{350};
t496 = ct{351};
t497 = ct{352};
t5 = ct{353};
t519 = ct{354};
t520 = ct{355};
t521 = ct{356};
t522 = ct{357};
t523 = ct{358};
t524 = ct{359};
t525 = ct{360};
t526 = ct{361};
t527 = ct{362};
t528 = ct{363};
t529 = ct{364};
t531 = ct{365};
t532 = ct{366};
t533 = ct{367};
t534 = ct{368};
t535 = ct{369};
t536 = ct{370};
t537 = ct{371};
t538 = ct{372};
t539 = ct{373};
t540 = ct{374};
t541 = ct{375};
t542 = ct{376};
t543 = ct{377};
t544 = ct{378};
t545 = ct{379};
t546 = ct{380};
t547 = ct{381};
t548 = ct{382};
t549 = ct{383};
t55 = ct{384};
t550 = ct{385};
t551 = ct{386};
t552 = ct{387};
t553 = ct{388};
t554 = ct{389};
t555 = ct{390};
t556 = ct{391};
t557 = ct{392};
t558 = ct{393};
t559 = ct{394};
t56 = ct{395};
t560 = ct{396};
t561 = ct{397};
t57 = ct{398};
t571 = ct{399};
t572 = ct{400};
t573 = ct{401};
t574 = ct{402};
t575 = ct{403};
t576 = ct{404};
t577 = ct{405};
t578 = ct{406};
t579 = ct{407};
t58 = ct{408};
t580 = ct{409};
t581 = ct{410};
t582 = ct{411};
t583 = ct{412};
t584 = ct{413};
t585 = ct{414};
t586 = ct{415};
t587 = ct{416};
t588 = ct{417};
t589 = ct{418};
t59 = ct{419};
t590 = ct{420};
t591 = ct{421};
t592 = ct{422};
t593 = ct{423};
t594 = ct{424};
t6 = ct{425};
t60 = ct{426};
t600 = ct{427};
t601 = ct{428};
t602 = ct{429};
t603 = ct{430};
t607 = ct{431};
t61 = ct{432};
t613 = ct{433};
t614 = ct{434};
t615 = ct{435};
t616 = ct{436};
t619 = ct{437};
t62 = ct{438};
t622 = ct{439};
t625 = ct{440};
t628 = ct{441};
t629 = ct{442};
t63 = ct{443};
t630 = ct{444};
t631 = ct{445};
t632 = ct{446};
t633 = ct{447};
t634 = ct{448};
t635 = ct{449};
t636 = ct{450};
t637 = ct{451};
t638 = ct{452};
t639 = ct{453};
t64 = ct{454};
t640 = ct{455};
t641 = ct{456};
t642 = ct{457};
t643 = ct{458};
t644 = ct{459};
t645 = ct{460};
t646 = ct{461};
t647 = ct{462};
t648 = ct{463};
t65 = ct{464};
t651 = ct{465};
t654 = ct{466};
t657 = ct{467};
t66 = ct{468};
t660 = ct{469};
t661 = ct{470};
t665 = ct{471};
t668 = ct{472};
t669 = ct{473};
t67 = ct{474};
t670 = ct{475};
t674 = ct{476};
t677 = ct{477};
t678 = ct{478};
t679 = ct{479};
t68 = ct{480};
t681 = ct{481};
t682 = ct{482};
t684 = ct{483};
t685 = ct{484};
t686 = ct{485};
t687 = ct{486};
t688 = ct{487};
t689 = ct{488};
t691 = ct{489};
t692 = ct{490};
t694 = ct{491};
t695 = ct{492};
t696 = ct{493};
t697 = ct{494};
t7 = ct{495};
t700 = ct{496};
t703 = ct{497};
t712 = ct{498};
t713 = ct{499};
t714 = ct{500};
t715 = ct{501};
t716 = ct{502};
t717 = ct{503};
t718 = ct{504};
t719 = ct{505};
t722 = ct{506};
t723 = ct{507};
t724 = ct{508};
t725 = ct{509};
t726 = ct{510};
t727 = ct{511};
t728 = ct{512};
t729 = ct{513};
t730 = ct{514};
t731 = ct{515};
t732 = ct{516};
t733 = ct{517};
t734 = ct{518};
t735 = ct{519};
t736 = ct{520};
t740 = ct{521};
t746 = ct{522};
t747 = ct{523};
t748 = ct{524};
t749 = ct{525};
t750 = ct{526};
t751 = ct{527};
t752 = ct{528};
t753 = ct{529};
t754 = ct{530};
t755 = ct{531};
t756 = ct{532};
t757 = ct{533};
t758 = ct{534};
t759 = ct{535};
t760 = ct{536};
t761 = ct{537};
t762 = ct{538};
t763 = ct{539};
t764 = ct{540};
t765 = ct{541};
t766 = ct{542};
t767 = ct{543};
t768 = ct{544};
t770 = ct{545};
t771 = ct{546};
t772 = ct{547};
t773 = ct{548};
t774 = ct{549};
t775 = ct{550};
t776 = ct{551};
t777 = ct{552};
t778 = ct{553};
t779 = ct{554};
t780 = ct{555};
t781 = ct{556};
t782 = ct{557};
t783 = ct{558};
t784 = ct{559};
t785 = ct{560};
t786 = ct{561};
t787 = ct{562};
t788 = ct{563};
t789 = ct{564};
t790 = ct{565};
t791 = ct{566};
t792 = ct{567};
t794 = ct{568};
t795 = ct{569};
t797 = ct{570};
t798 = ct{571};
t8 = ct{572};
t800 = ct{573};
t801 = ct{574};
t803 = ct{575};
t804 = ct{576};
t805 = ct{577};
t806 = ct{578};
t816 = ct{579};
t818 = ct{580};
t82 = ct{581};
t820 = ct{582};
t822 = ct{583};
t823 = ct{584};
t825 = ct{585};
t827 = ct{586};
t829 = ct{587};
t83 = ct{588};
t831 = ct{589};
t832 = ct{590};
t833 = ct{591};
t834 = ct{592};
t852 = ct{593};
t855 = ct{594};
t858 = ct{595};
t861 = ct{596};
t864 = ct{597};
t865 = ct{598};
t866 = ct{599};
t867 = ct{600};
t868 = ct{601};
t869 = ct{602};
t870 = ct{603};
t871 = ct{604};
t872 = ct{605};
t873 = ct{606};
t874 = ct{607};
t875 = ct{608};
t876 = ct{609};
t877 = ct{610};
t878 = ct{611};
t879 = ct{612};
t881 = ct{613};
t883 = ct{614};
t885 = ct{615};
t887 = ct{616};
t888 = ct{617};
t889 = ct{618};
t890 = ct{619};
t891 = ct{620};
t9 = ct{621};
t900 = ct{622};
t902 = ct{623};
t903 = ct{624};
t904 = ct{625};
t906 = ct{626};
t907 = ct{627};
t908 = ct{628};
t910 = ct{629};
t911 = ct{630};
t912 = ct{631};
t914 = ct{632};
t915 = ct{633};
t916 = ct{634};
t917 = ct{635};
t918 = ct{636};
t919 = ct{637};
t920 = ct{638};
t921 = ct{639};
t922 = ct{640};
t923 = ct{641};
t924 = ct{642};
t925 = ct{643};
t926 = ct{644};
t927 = ct{645};
t93 = ct{646};
t930 = ct{647};
t94 = ct{648};
t943 = ct{649};
t944 = ct{650};
t945 = ct{651};
t946 = ct{652};
t947 = ct{653};
t948 = ct{654};
t949 = ct{655};
t950 = ct{656};
t951 = ct{657};
t953 = ct{658};
t955 = ct{659};
t957 = ct{660};
t959 = ct{661};
t960 = ct{662};
t961 = ct{663};
t962 = ct{664};
t963 = ct{665};
t964 = ct{666};
t965 = ct{667};
t966 = ct{668};
t967 = ct{669};
t968 = ct{670};
t969 = ct{671};
t970 = ct{672};
t971 = ct{673};
t972 = ct{674};
t973 = ct{675};
t974 = ct{676};
t977 = ct{677};
t979 = ct{678};
t980 = ct{679};
t982 = ct{680};
t984 = ct{681};
t985 = ct{682};
t986 = ct{683};
t987 = ct{684};
t988 = ct{685};
t989 = ct{686};
t990 = ct{687};
t991 = ct{688};
t993 = ct{689};
t995 = ct{690};
t997 = ct{691};
t999 = ct{692};
t807 = -t722;
t808 = -t723;
t809 = -t724;
t810 = -t725;
t811 = -t730;
t812 = -t732;
t813 = -t733;
t814 = -t735;
t844 = t172.*(3.3e+1./1.0e+3);
t845 = t173.*(3.3e+1./1.0e+3);
t846 = t174.*(3.3e+1./1.0e+3);
t847 = t175.*(3.3e+1./1.0e+3);
t848 = t176.*(5.1e+1./1.0e+3);
t849 = t177.*(5.1e+1./1.0e+3);
t850 = t178.*(5.1e+1./1.0e+3);
t851 = t179.*(5.1e+1./1.0e+3);
t853 = -t794;
t854 = -t795;
t856 = -t797;
t857 = -t798;
t859 = -t800;
t860 = -t801;
t862 = -t803;
t863 = -t804;
t892 = t94.*t383;
t893 = t94.*t385;
t894 = t94.*t389;
t895 = t94.*t391;
t896 = t94.*t395;
t897 = t94.*t397;
t898 = t94.*t401;
t899 = t94.*t403;
t928 = t171.*4.033333333333333e-2;
t929 = t171.*4.366666666666667e-2;
t935 = -t864;
t936 = -t867;
t937 = -t868;
t938 = -t871;
t939 = -t873;
t940 = -t874;
t941 = -t877;
t942 = -t878;
t952 = -t902;
t954 = -t906;
t956 = -t910;
t958 = -t914;
t992 = t3.*t94.*t437;
t994 = t3.*t94.*t438;
t996 = t3.*t94.*t440;
t998 = t3.*t94.*t441;
t1000 = t3.*t94.*t443;
t1002 = t3.*t94.*t444;
t1004 = t3.*t94.*t446;
t1006 = t3.*t94.*t447;
t1008 = -t960;
t1009 = -t962;
t1010 = -t964;
t1011 = -t966;
t1018 = t2.*t16.*t461.*(2.0./5.0);
t1019 = t2.*t16.*t464.*(2.0./5.0);
t1020 = t2.*t16.*t467.*(2.0./5.0);
t1021 = t2.*t16.*t470.*(2.0./5.0);
t1022 = -t985;
t1023 = -t987;
t1024 = -t989;
t1025 = -t991;
t1038 = t16.*t17.*t461.*(2.0./5.0);
t1039 = t16.*t17.*t464.*(2.0./5.0);
t1040 = t16.*t17.*t467.*(2.0./5.0);
t1041 = t16.*t17.*t470.*(2.0./5.0);
t1043 = -t995;
t1045 = -t999;
t1047 = -t1003;
t1049 = -t1007;
t1137 = -t1085;
t1138 = -t1087;
t1139 = -t1089;
t1140 = -t1091;
t1153 = -t1109;
t1154 = -t1111;
t1155 = -t1113;
t1156 = -t1115;
t1182 = t171.*t172.*(3.3e+1./5.0e+2);
t1183 = t171.*t173.*(3.3e+1./5.0e+2);
t1184 = t171.*t174.*(3.3e+1./5.0e+2);
t1185 = t171.*t175.*(3.3e+1./5.0e+2);
t1186 = t171.*t176.*(5.1e+1./5.0e+2);
t1187 = t171.*t177.*(5.1e+1./5.0e+2);
t1188 = t171.*t178.*(5.1e+1./5.0e+2);
t1189 = t171.*t179.*(5.1e+1./5.0e+2);
t1220 = t121.*t131.*t171.*(3.0./2.5e+2);
t1221 = t122.*t132.*t171.*(3.0./2.5e+2);
t1222 = t123.*t133.*t171.*(3.0./2.5e+2);
t1223 = t124.*t134.*t171.*(3.0./2.5e+2);
t1224 = t125.*t135.*t171.*(3.0./2.5e+2);
t1225 = t126.*t136.*t171.*(3.0./2.5e+2);
t1226 = t127.*t137.*t171.*(3.0./2.5e+2);
t1227 = t128.*t138.*t171.*(3.0./2.5e+2);
t1241 = t21.*t1083.*(3.0./5.0e+1);
t1243 = t24.*t1083.*(3.0./5.0e+1);
t1245 = t27.*t1083.*(3.0./5.0e+1);
t1247 = t30.*t1083.*(3.0./5.0e+1);
t1261 = -t1254;
t1262 = -t1255;
t1263 = -t1256;
t1264 = -t1257;
t1292 = t94.*t1252;
t1293 = t94.*t1253;
t1294 = t94.*t1254;
t1295 = t94.*t1255;
t1296 = t94.*t1256;
t1297 = t94.*t1257;
t1298 = t94.*t1258;
t1299 = t94.*t1259;
t1308 = t462.*t1082.*(2.0./5.0);
t1309 = t465.*t1082.*(2.0./5.0);
t1310 = t468.*t1082.*(2.0./5.0);
t1311 = t471.*t1082.*(2.0./5.0);
t1345 = t169+t209+t222+t547;
t1346 = t169+t226+t289+t415;
t1347 = t169+t228+t290+t548;
t1374 = t325+t330+t607+t740;
t1375 = t328+t330+t613+t746;
t1376 = t255+t473+t748+t832;
t1377 = t258+t473+t749+t833;
t1378 = t324+t473+t747+t831;
t1379 = t327+t473+t750+t834;
t1384 = t233+t357+t381+t496+t661;
t1393 = t233+t363+t399+t574+t670;
t1399 = t233+t361+t533+t572+t771;
t1400 = t306+t383+t561+t576+t685+t774+t823+t900+t1014;
t1403 = t306+t401+t561+t588+t782+t790+t829+t912+t982;
t1408 = t93+t108+t109+t110+t111+t112+t113+t114+t115+t116+t117+t118+t119+t263+t265+t267+t269+t433+t434+t435+t436;
t1418 = t104+t105+t106+t107+t142+t144+t145+t146+t147+t148+t149+t150+t151+t180+t181+t182+t183+t184+t185+t186+t187+t188+t189+t190+t191+t426+t428+t430+t432+t600+t601+t602+t603;
t348 = -t271;
t349 = -t272;
t570 = -t490;
t737 = t82+t193;
t738 = t83+t192;
t931 = -t844;
t932 = -t845;
t933 = -t846;
t934 = -t847;
t975 = -t929;
t1012 = t129+t560;
t1013 = t139+t555;
t1026 = t4.*t554.*(3.0./5.0e+1);
t1027 = t5.*t554.*(3.0./5.0e+1);
t1028 = t6.*t554.*(3.0./5.0e+1);
t1029 = t7.*t554.*(3.0./5.0e+1);
t1030 = t8.*t554.*(3.0./5.0e+1);
t1031 = t9.*t554.*(3.0./5.0e+1);
t1032 = t10.*t554.*(3.0./5.0e+1);
t1033 = t11.*t554.*(3.0./5.0e+1);
t1034 = t12.*t554.*(3.0./5.0e+1);
t1035 = t13.*t554.*(3.0./5.0e+1);
t1036 = t14.*t554.*(3.0./5.0e+1);
t1037 = t15.*t554.*(3.0./5.0e+1);
t1050 = t19.*t553.*(3.0./5.0e+1);
t1051 = t19.*t554.*(3.0./5.0e+1);
t1052 = t20.*t553.*(3.0./5.0e+1);
t1053 = t20.*t554.*(3.0./5.0e+1);
t1054 = t21.*t553.*(3.0./5.0e+1);
t1055 = t21.*t554.*(3.0./5.0e+1);
t1056 = t22.*t553.*(3.0./5.0e+1);
t1057 = t22.*t554.*(3.0./5.0e+1);
t1058 = t23.*t553.*(3.0./5.0e+1);
t1059 = t23.*t554.*(3.0./5.0e+1);
t1060 = t24.*t553.*(3.0./5.0e+1);
t1061 = t24.*t554.*(3.0./5.0e+1);
t1062 = t25.*t553.*(3.0./5.0e+1);
t1063 = t25.*t554.*(3.0./5.0e+1);
t1064 = t26.*t553.*(3.0./5.0e+1);
t1065 = t26.*t554.*(3.0./5.0e+1);
t1066 = t27.*t553.*(3.0./5.0e+1);
t1067 = t27.*t554.*(3.0./5.0e+1);
t1068 = t28.*t553.*(3.0./5.0e+1);
t1069 = t28.*t554.*(3.0./5.0e+1);
t1070 = t29.*t553.*(3.0./5.0e+1);
t1071 = t29.*t554.*(3.0./5.0e+1);
t1072 = t30.*t553.*(3.0./5.0e+1);
t1073 = t30.*t554.*(3.0./5.0e+1);
t1104 = -t1038;
t1105 = -t1039;
t1106 = -t1040;
t1107 = -t1041;
t1132 = (t94.*t553)./2.0;
t1215 = -t1186;
t1216 = -t1187;
t1217 = -t1188;
t1218 = -t1189;
t1228 = -t1220;
t1229 = -t1221;
t1230 = -t1222;
t1231 = -t1223;
t1232 = -t1224;
t1233 = -t1225;
t1234 = -t1226;
t1235 = -t1227;
t1248 = -t1241;
t1249 = -t1243;
t1250 = -t1245;
t1251 = -t1247;
t1272 = (t94.*t462.*t554)./5.0;
t1273 = (t94.*t463.*t554)./5.0;
t1274 = (t94.*t465.*t554)./5.0;
t1275 = (t94.*t466.*t554)./5.0;
t1276 = (t94.*t468.*t554)./5.0;
t1277 = (t94.*t469.*t554)./5.0;
t1278 = (t94.*t471.*t554)./5.0;
t1279 = (t94.*t472.*t554)./5.0;
t1401 = t306+t531+t561+t580+t679+t695+t825+t904+t1015;
t1402 = t306+t534+t561+t584+t689+t786+t827+t908+t980;
t1404 = t306+t385+t578+t614+t687+t776+t916+t952+t977;
t1405 = t306+t532+t582+t614+t682+t697+t917+t954+t979;
t1406 = t306+t535+t586+t614+t692+t788+t918+t956+t1016;
t1407 = t306+t403+t590+t614+t784+t792+t919+t958+t1017;
t1409 = t16.*t1408.*(3.0./1.0e+2);
t1419 = t2.*t1418.*(3.0./1.0e+2);
t1420 = t17.*t1418.*(3.0./1.0e+2);
t1428 = t237+t238+t294+t295+t296+t297+t298+t299+t300+t301+t302+t303+t304+t305+t309+t310+t365+t366+t368+t369+t374+t375+t421+t422+t423+t424+t450+t451+t453+t454+t456+t457+t459+t460+t519+t520+t521+t522+t523+t524+t549+t550+t551+t552+t556+t557+t558+t559+t729+t731+t734+t736+t811+t812+t813+t814+t959+t961+t963+t965+t1008+t1009+t1010+t1011;
t1429 = t311+t312+t313+t314+t315+t316+t317+t318+t319+t320+t321+t322+t437+t438+t439+t440+t441+t442+t443+t444+t445+t446+t447+t448+t486+t487+t488+t489+t495+t497+t539+t540+t541+t542+t543+t544+t545+t546+t571+t573+t616+t619+t622+t625+t640+t641+t642+t643+t644+t645+t646+t647+t665+t668+t674+t677+t684+t686+t694+t696+t700+t703+t716+t751+t752+t753+t754+t755+t756+t757+t758+t767+t772+t777+t778+t779+t780+t785+t787+t789+t791+t865+t869+t875+t879+t893+t894+t896+t899+t936+t938+t939+t941+t947+t948+t949+t950+t993+t997+t1001+t1005+t1043+t1045+t1047+t1049;
t1430 = t356+t358+t360+t362+t377+t378+t388+t390+t392+t394+t396+t398+t525+t526+t527+t528+t529+t536+t537+t538+t575+t577+t579+t581+t583+t585+t587+t589+t591+t592+t593+t594+t628+t629+t630+t631+t632+t633+t634+t635+t636+t637+t638+t639+t648+t651+t654+t657+t660+t669+t678+t681+t688+t691+t712+t713+t714+t715+t717+t718+t719+t726+t727+t728+t759+t760+t761+t762+t763+t764+t765+t766+t768+t770+t773+t775+t781+t783+t805+t806+t807+t808+t809+t810+t816+t818+t820+t822+t852+t853+t854+t855+t856+t857+t858+t859+t860+t861+t862+t863+t866+t870+t872+t876+t881+t883+t885+t887+t888+t889+t890+t891+t903+t907+t911+t915+t920+t921+t922+t923+t924+t925+t926+t927+t930+t935+t937+t940+t942+t943+t944+t945+t946+t951+t953+t955+t957+t984+t986+t988+t990+t994+t998+t1002+t1006+t1022+t1023+t1024+t1025+t1042+t1044+t1046+t1048+t1075+t1076+t1078+t1081+t1084+t1086+t1088+t1090+t1108+t1110+t1112+t1114+t1128+t1129+t1130+t1131+t1137+t1138+t1139+t1140+t1153+t1154+t1155+t1156;
t1092 = -t1026;
t1093 = -t1027;
t1094 = -t1028;
t1095 = -t1029;
t1096 = -t1030;
t1097 = -t1031;
t1098 = -t1032;
t1099 = -t1033;
t1100 = -t1034;
t1101 = -t1035;
t1102 = -t1036;
t1103 = -t1037;
t1116 = -t1051;
t1117 = -t1053;
t1118 = -t1055;
t1119 = -t1057;
t1120 = -t1059;
t1121 = -t1061;
t1122 = -t1063;
t1123 = -t1065;
t1124 = -t1067;
t1125 = -t1069;
t1126 = -t1071;
t1127 = -t1073;
t1141 = t4.*t737.*(3.0./5.0e+1);
t1142 = t5.*t737.*(3.0./5.0e+1);
t1143 = t6.*t737.*(3.0./5.0e+1);
t1144 = t7.*t737.*(3.0./5.0e+1);
t1145 = t8.*t737.*(3.0./5.0e+1);
t1146 = t9.*t737.*(3.0./5.0e+1);
t1147 = t10.*t737.*(3.0./5.0e+1);
t1148 = t11.*t737.*(3.0./5.0e+1);
t1149 = t12.*t737.*(3.0./5.0e+1);
t1150 = t13.*t737.*(3.0./5.0e+1);
t1151 = t14.*t737.*(3.0./5.0e+1);
t1152 = t15.*t737.*(3.0./5.0e+1);
t1157 = t19.*t737.*(3.0./5.0e+1);
t1158 = t19.*t738.*(3.0./5.0e+1);
t1159 = t20.*t737.*(3.0./5.0e+1);
t1160 = t20.*t738.*(3.0./5.0e+1);
t1161 = t21.*t737.*(3.0./5.0e+1);
t1162 = t21.*t738.*(3.0./5.0e+1);
t1163 = t22.*t737.*(3.0./5.0e+1);
t1164 = t22.*t738.*(3.0./5.0e+1);
t1165 = t23.*t737.*(3.0./5.0e+1);
t1166 = t23.*t738.*(3.0./5.0e+1);
t1167 = t24.*t737.*(3.0./5.0e+1);
t1168 = t24.*t738.*(3.0./5.0e+1);
t1169 = t25.*t737.*(3.0./5.0e+1);
t1170 = t25.*t738.*(3.0./5.0e+1);
t1171 = t26.*t737.*(3.0./5.0e+1);
t1172 = t26.*t738.*(3.0./5.0e+1);
t1173 = t27.*t737.*(3.0./5.0e+1);
t1174 = t27.*t738.*(3.0./5.0e+1);
t1175 = t28.*t737.*(3.0./5.0e+1);
t1176 = t28.*t738.*(3.0./5.0e+1);
t1177 = t29.*t737.*(3.0./5.0e+1);
t1178 = t29.*t738.*(3.0./5.0e+1);
t1179 = t30.*t737.*(3.0./5.0e+1);
t1180 = t30.*t738.*(3.0./5.0e+1);
t1181 = -t1132;
t1214 = (t94.*t738)./2.0;
t1236 = t20.*t1013.*(3.0./5.0e+1);
t1237 = t23.*t1013.*(3.0./5.0e+1);
t1238 = t26.*t1013.*(3.0./5.0e+1);
t1239 = t29.*t1013.*(3.0./5.0e+1);
t1260 = t167+t1132;
t1284 = -t1273;
t1285 = -t1275;
t1286 = -t1277;
t1287 = -t1279;
t1288 = t463.*t1012.*(2.0./5.0);
t1289 = t466.*t1012.*(2.0./5.0);
t1290 = t469.*t1012.*(2.0./5.0);
t1291 = t472.*t1012.*(2.0./5.0);
t1300 = (t94.*t462.*t737)./5.0;
t1301 = (t94.*t463.*t737)./5.0;
t1302 = (t94.*t465.*t737)./5.0;
t1303 = (t94.*t466.*t737)./5.0;
t1304 = (t94.*t468.*t737)./5.0;
t1305 = (t94.*t469.*t737)./5.0;
t1306 = (t94.*t471.*t737)./5.0;
t1307 = (t94.*t472.*t737)./5.0;
t1341 = t476+t1248;
t1342 = t479+t1249;
t1343 = t482+t1250;
t1344 = t485+t1251;
t1410 = t931+t967+t975+t1182+t1228+t1252+t1292+2.183333333333333e-2;
t1411 = t851+t928+t974+t1218+t1235+t1259+t1299-2.016666666666667e-2;
t1412 = t932+t968+t975+t1183+t1229+t1253+t1312+2.183333333333333e-2;
t1413 = t933+t969+t975+t1184+t1230+t1261+t1294+2.183333333333333e-2;
t1414 = t849+t928+t972+t1216+t1233+t1264+t1297-2.016666666666667e-2;
t1415 = t850+t928+t973+t1217+t1234+t1258+t1315-2.016666666666667e-2;
t1416 = t934+t970+t975+t1185+t1231+t1262+t1313+2.183333333333333e-2;
t1417 = t848+t928+t971+t1215+t1232+t1263+t1314-2.016666666666667e-2;
t1421 = -t1419;
t1422 = -t1420;
t1190 = -t1157;
t1191 = -t1158;
t1192 = -t1159;
t1193 = -t1160;
t1194 = -t1161;
t1195 = -t1162;
t1196 = -t1163;
t1197 = -t1164;
t1198 = -t1165;
t1199 = -t1166;
t1200 = -t1167;
t1201 = -t1168;
t1202 = -t1169;
t1203 = -t1170;
t1204 = -t1171;
t1205 = -t1172;
t1206 = -t1173;
t1207 = -t1174;
t1208 = -t1175;
t1209 = -t1176;
t1210 = -t1177;
t1211 = -t1178;
t1212 = -t1179;
t1213 = -t1180;
t1219 = -t1214;
t1240 = -t1236;
t1242 = -t1237;
t1244 = -t1238;
t1246 = -t1239;
t1265 = t167+t1181;
t1266 = t166+t1214;
t1267 = t491+t1092;
t1268 = t492+t1095;
t1269 = t493+t1098;
t1270 = t494+t1101;
t1280 = t352+t1141;
t1281 = t353+t1144;
t1282 = t354+t1147;
t1283 = t355+t1150;
t1316 = -t1300;
t1317 = -t1302;
t1318 = -t1304;
t1319 = -t1306;
t1320 = t21.*t1260.*(3.0./5.0e+1);
t1321 = t24.*t1260.*(3.0./5.0e+1);
t1322 = t27.*t1260.*(3.0./5.0e+1);
t1323 = t30.*t1260.*(3.0./5.0e+1);
t1348 = t463.*t1260.*(2.0./5.0);
t1349 = t466.*t1260.*(2.0./5.0);
t1350 = t469.*t1260.*(2.0./5.0);
t1351 = t472.*t1260.*(2.0./5.0);
t1423 = t170+t214+t215+t216+t217+t231+t277+t278+t279+t280+t281+t282+t283+t284+t285+t286+t287+t288+t1288+t1289+t1290+t1291+t1308+t1309+t1310+t1311;
t1271 = t166+t1219;
t1324 = t20.*t1265.*(3.0./5.0e+1);
t1325 = t23.*t1265.*(3.0./5.0e+1);
t1326 = t26.*t1265.*(3.0./5.0e+1);
t1327 = t29.*t1265.*(3.0./5.0e+1);
t1328 = t20.*t1266.*(3.0./5.0e+1);
t1329 = t23.*t1266.*(3.0./5.0e+1);
t1330 = t26.*t1266.*(3.0./5.0e+1);
t1331 = t29.*t1266.*(3.0./5.0e+1);
t1332 = t475+t1240;
t1333 = t478+t1242;
t1334 = t481+t1244;
t1335 = t484+t1246;
t1352 = t462.*t1265.*(2.0./5.0);
t1353 = t465.*t1265.*(2.0./5.0);
t1354 = t468.*t1265.*(2.0./5.0);
t1355 = t471.*t1265.*(2.0./5.0);
t1356 = t462.*t1266.*(2.0./5.0);
t1357 = t465.*t1266.*(2.0./5.0);
t1358 = t468.*t1266.*(2.0./5.0);
t1359 = t471.*t1266.*(2.0./5.0);
t1380 = t1143+t1320;
t1381 = t1146+t1321;
t1382 = t1149+t1322;
t1383 = t1152+t1323;
t1424 = t208+t376+t1050+t1052+t1054+t1056+t1058+t1060+t1062+t1064+t1066+t1068+t1070+t1072+t1301+t1303+t1305+t1307+t1316+t1317+t1318+t1319;
t1425 = t293+t350+t1191+t1193+t1195+t1197+t1199+t1201+t1203+t1205+t1207+t1209+t1211+t1213+t1272+t1274+t1276+t1278+t1284+t1285+t1286+t1287;
t1337 = t21.*t1271.*(3.0./5.0e+1);
t1338 = t24.*t1271.*(3.0./5.0e+1);
t1339 = t27.*t1271.*(3.0./5.0e+1);
t1340 = t30.*t1271.*(3.0./5.0e+1);
t1360 = -t1356;
t1361 = t463.*t1271.*(2.0./5.0);
t1362 = -t1357;
t1363 = t466.*t1271.*(2.0./5.0);
t1364 = -t1358;
t1365 = t469.*t1271.*(2.0./5.0);
t1366 = -t1359;
t1367 = t472.*t1271.*(2.0./5.0);
t1385 = t1093+t1328;
t1386 = t1096+t1329;
t1387 = t1099+t1330;
t1388 = t1102+t1331;
t1389 = t1142+t1324;
t1390 = t1145+t1325;
t1391 = t1148+t1326;
t1392 = t1151+t1327;
t1427 = t292+t351+t1104+t1105+t1106+t1107+t1190+t1192+t1194+t1196+t1198+t1200+t1202+t1204+t1206+t1208+t1210+t1212+t1348+t1349+t1350+t1351+t1352+t1353+t1354+t1355;
t1370 = -t1361;
t1371 = -t1363;
t1372 = -t1365;
t1373 = -t1367;
t1394 = t1094+t1337;
t1395 = t1097+t1338;
t1396 = t1100+t1339;
t1397 = t1103+t1340;
t1426 = t308+t570+t1018+t1019+t1020+t1021+t1116+t1117+t1118+t1119+t1120+t1121+t1122+t1123+t1124+t1125+t1126+t1127+t1360+t1362+t1364+t1366+t1370+t1371+t1372+t1373;
et1 = (t195+t203+t219+t272+t343+t25.*t554.*(3.0./2.0e+1)-t2.*t16.*t467).^2.*(2.0./5.0)+(t203+t213+t219+t272+t343+t22.*t554.*(3.0./2.0e+1)-t2.*t16.*t464).^2.*(2.0./5.0)+(t195+t201+t203+t343+t349+t28.*t554.*(3.0./2.0e+1)-t2.*t16.*t470).^2.*(2.0./5.0)+(t201+t203+t213+t343+t349+t19.*t554.*(3.0./2.0e+1)-t2.*t16.*t461).^2.*(2.0./5.0)+(t194+t202+t218+t271+t291-t25.*t737.*(3.0./2.0e+1)-t16.*t17.*t467).^2.*(2.0./5.0)+(t194+t200+t202+t291+t348+t19.*t737.*(3.0./2.0e+1)+t16.*t17.*t461).^2.*(2.0./5.0)+(t194+t200+t230+t291+t348+t28.*t737.*(3.0./2.0e+1)+t16.*t17.*t470).^2.*(2.0./5.0);
et2 = (t19.*t31-t3.*t4.*t16).*((t19.*t31)./6.0e+2-(t3.*t4.*t16)./6.0e+2)+(t22.*t31-t3.*t7.*t16).*((t22.*t31)./6.0e+2-(t3.*t7.*t16)./6.0e+2)+(t25.*t31-t3.*t10.*t16).*((t25.*t31)./6.0e+2-(t3.*t10.*t16)./6.0e+2)+(t28.*t31-t3.*t13.*t16).*((t28.*t31)./6.0e+2-(t3.*t13.*t16)./6.0e+2)+(t20.*t1013+t3.*t5.*t16).*((t20.*t1013)./6.0e+2+(t3.*t5.*t16)./6.0e+2)+(t23.*t1013+t3.*t8.*t16).*((t23.*t1013)./6.0e+2+(t3.*t8.*t16)./6.0e+2);
et3 = (t26.*t1013+t3.*t11.*t16).*((t26.*t1013)./6.0e+2+(t3.*t11.*t16)./6.0e+2)+(t29.*t1013+t3.*t14.*t16).*((t29.*t1013)./6.0e+2+(t3.*t14.*t16)./6.0e+2)+(t21.*t1083+t3.*t6.*t16).*((t21.*t1083)./6.0e+2+(t3.*t6.*t16)./6.0e+2)+(t24.*t1083+t3.*t9.*t16).*((t24.*t1083)./6.0e+2+(t3.*t9.*t16)./6.0e+2)+(t27.*t1083+t3.*t12.*t16).*((t27.*t1083)./6.0e+2+(t3.*t12.*t16)./6.0e+2)+(t30.*t1083+t3.*t15.*t16).*((t30.*t1083)./6.0e+2+(t3.*t15.*t16)./6.0e+2)+t46.*t67.*6.0025e-2;
et4 = (t195+t203+t219+t272+t343+t26.*t554.*(3.0./2.0e+1)+t468.*t1266).^2.*(2.0./5.0)+(t195+t203+t219+t272+t343+t27.*t554.*(3.0./2.0e+1)+t469.*t1271).^2.*(2.0./5.0)+(t203+t213+t219+t272+t343+t23.*t554.*(3.0./2.0e+1)+t465.*t1266).^2.*(2.0./5.0)+(t203+t213+t219+t272+t343+t24.*t554.*(3.0./2.0e+1)+t466.*t1271).^2.*(2.0./5.0)+(t195+t201+t203+t343+t349+t29.*t554.*(3.0./2.0e+1)+t471.*t1266).^2.*(2.0./5.0)+(t201+t203+t213+t343+t349+t20.*t554.*(3.0./2.0e+1)+t462.*t1266).^2.*(2.0./5.0)+(t195+t201+t203+t343+t349+t30.*t554.*(3.0./2.0e+1)+t472.*t1271).^2.*(2.0./5.0)+(t201+t203+t213+t343+t349+t21.*t554.*(3.0./2.0e+1)+t463.*t1271).^2.*(2.0./5.0)+(t194+t202+t218+t271+t291-t27.*t737.*(3.0./2.0e+1)+t469.*t1260).^2.*(2.0./5.0);
et5 = (t194+t202+t218+t271+t291-t26.*t737.*(3.0./2.0e+1)+t468.*t1265).^2.*(2.0./5.0)+(t194+t218+t230+t271+t291-t24.*t737.*(3.0./2.0e+1)+t466.*t1260).^2.*(2.0./5.0)+(t194+t218+t230+t271+t291-t23.*t737.*(3.0./2.0e+1)+t465.*t1265).^2.*(2.0./5.0)+(t194+t200+t202+t291+t348+t21.*t737.*(3.0./2.0e+1)-t463.*t1260).^2.*(2.0./5.0)+(t194+t200+t202+t291+t348+t20.*t737.*(3.0./2.0e+1)-t462.*t1265).^2.*(2.0./5.0)+(t194+t200+t230+t291+t348+t30.*t737.*(3.0./2.0e+1)-t472.*t1260).^2.*(2.0./5.0)+(t194+t200+t230+t291+t348+t29.*t737.*(3.0./2.0e+1)-t471.*t1265).^2.*(2.0./5.0)+t18.^2.*t67.*1.156666666666667e-2+(t168-t329).*(t307-t615).*4.0;
et6 = (-t194+t200+t202-t291+t348+t22.*t737.*(3.0./2.0e+1)+t16.*t17.*t464).^2.*(2.0./5.0)+t31.^2.*4.9e-3+(t168+t329).*(t307+t615).*4.0;
et7 = t4.*(3.0./5.0e+1)-t5.*9.75e-3-t6.*9.75e-3+t7.*(3.0./5.0e+1)-t8.*9.75e-3-t9.*9.75e-3-t10.*(3.0./1.25e+2)+t11.*3.225e-2+t12.*3.225e-2-t13.*(3.0./1.25e+2)+t14.*3.225e-2+t15.*3.225e-2+t19.*(3.0./5.0e+2)+t20.*(3.0./5.0e+2)+t21.*(3.0./5.0e+2)+t22.*(3.0./5.0e+2)+t23.*(3.0./5.0e+2)+t24.*(3.0./5.0e+2)+t25.*(3.0./5.0e+2)+t26.*(3.0./5.0e+2)+t27.*(3.0./5.0e+2)+t28.*(3.0./5.0e+2)+t29.*(3.0./5.0e+2)+t30.*(3.0./5.0e+2);
et8 = t45.*(-2.605625e-1)+t55.*(2.0./3.75e+2)+t56./7.5e+2+t57./7.5e+2+t58.*(2.0./3.75e+2)+t59./7.5e+2+t60./7.5e+2+t61.*(2.0./3.75e+2)+t62./7.5e+2+t63./7.5e+2+t64.*(2.0./3.75e+2)+t65./7.5e+2+t66./7.5e+2-t5.*t45.*6.75e-3-t6.*t45.*6.75e-3-t8.*t45.*6.75e-3-t9.*t45.*6.75e-3-t11.*t45.*6.75e-3-t12.*t45.*6.75e-3-t14.*t45.*6.75e-3-t15.*t45.*6.75e-3;
et9 = t19.*t45.*(3.0./5.0e+2)+t20.*t45.*(3.0./5.0e+2)+t21.*t45.*(3.0./5.0e+2)+t22.*t45.*(3.0./5.0e+2)+t23.*t45.*(3.0./5.0e+2)+t24.*t45.*(3.0./5.0e+2)+t25.*t45.*(3.0./5.0e+2)+t26.*t45.*(3.0./5.0e+2)+t27.*t45.*(3.0./5.0e+2)+t28.*t45.*(3.0./5.0e+2)+t29.*t45.*(3.0./5.0e+2)+t30.*t45.*(3.0./5.0e+2)-t19.*t68.*(2.1e+1./1.0e+3)-t20.*t68.*(2.1e+1./1.0e+3)-t21.*t68.*(2.1e+1./1.0e+3)+t22.*t68.*(2.1e+1./1.0e+3)+t23.*t68.*(2.1e+1./1.0e+3)+t24.*t68.*(2.1e+1./1.0e+3)+t25.*t68.*(2.1e+1./1.0e+3)+t26.*t68.*(2.1e+1./1.0e+3)+t27.*t68.*(2.1e+1./1.0e+3)-t28.*t68.*(2.1e+1./1.0e+3);
et10 = t29.*t68.*(-2.1e+1./1.0e+3)-t30.*t68.*(2.1e+1./1.0e+3)+t5.*t94.*1.05e-2-t6.*t94.*1.05e-2-t45.*t55.*(2.0./3.75e+2)-t45.*t56.*(7.0./7.5e+2)-t8.*t94.*1.05e-2-t45.*t57.*(7.0./7.5e+2)+t9.*t94.*1.05e-2-t45.*t58.*(2.0./3.75e+2)-t45.*t59.*(7.0./7.5e+2)-t11.*t94.*1.05e-2-t45.*t60.*(7.0./7.5e+2)+t12.*t94.*1.05e-2-t45.*t61.*(2.0./3.75e+2)-t45.*t62.*(7.0./7.5e+2)+t14.*t94.*1.05e-2-t45.*t63.*(7.0./7.5e+2)-t15.*t94.*1.05e-2;
et11 = t45.*t64.*(-2.0./3.75e+2)-t45.*t65.*(7.0./7.5e+2)-t45.*t66.*(7.0./7.5e+2)-t5.*t45.*t94.*1.05e-2+t6.*t45.*t94.*1.05e-2+t8.*t45.*t94.*1.05e-2-t9.*t45.*t94.*1.05e-2+t11.*t45.*t94.*1.05e-2-t12.*t45.*t94.*1.05e-2-t14.*t45.*t94.*1.05e-2+t15.*t45.*t94.*1.05e-2-t5.*t68.*t94.*(3.0./1.0e+3)+t6.*t68.*t94.*(3.0./1.0e+3)-t8.*t68.*t94.*(3.0./1.0e+3)+t9.*t68.*t94.*(3.0./1.0e+3)-t11.*t68.*t94.*(3.0./1.0e+3)+t12.*t68.*t94.*(3.0./1.0e+3)-t14.*t68.*t94.*(3.0./1.0e+3);
et12 = t15.*t68.*t94.*(3.0./1.0e+3)-t20.*t68.*t94.*4.5e-3+t21.*t68.*t94.*4.5e-3-t23.*t68.*t94.*4.5e-3+t24.*t68.*t94.*4.5e-3-t26.*t68.*t94.*4.5e-3+t27.*t68.*t94.*4.5e-3-t29.*t68.*t94.*4.5e-3+t30.*t68.*t94.*4.5e-3-t5.*t20.*t68.*t94.*(2.0./3.75e+2)-t8.*t23.*t68.*t94.*(2.0./3.75e+2)-t11.*t26.*t68.*t94.*(2.0./3.75e+2)-t14.*t29.*t68.*t94.*(2.0./3.75e+2)+t6.*t21.*t68.*t330+t9.*t24.*t68.*t330+t12.*t27.*t68.*t330+t15.*t30.*t68.*t330+1.0834625;
et13 = t5.*1.35e-2+t6.*1.35e-2+t8.*1.35e-2+t9.*1.35e-2+t11.*1.35e-2+t12.*1.35e-2+t14.*1.35e-2+t15.*1.35e-2+t19.*(3.0./2.5e+2)+t20.*(3.0./2.5e+2)+t21.*(3.0./2.5e+2)+t22.*(3.0./2.5e+2)+t23.*(3.0./2.5e+2)+t24.*(3.0./2.5e+2)+t25.*(3.0./2.5e+2)+t26.*(3.0./2.5e+2)+t27.*(3.0./2.5e+2)+t28.*(3.0./2.5e+2)+t29.*(3.0./2.5e+2)+t30.*(3.0./2.5e+2)-t55.*(4.0./3.75e+2)-t56./3.75e+2-t57./3.75e+2-t58.*(4.0./3.75e+2)-t59./3.75e+2;
et14 = t60.*(-1.0./3.75e+2)-t61.*(4.0./3.75e+2)-t62./3.75e+2-t63./3.75e+2-t64.*(4.0./3.75e+2)-t65./3.75e+2-t66./3.75e+2-t6.*t94.*(2.1e+1./1.0e+3)-t8.*t94.*(2.1e+1./1.0e+3)-t11.*t94.*(2.1e+1./1.0e+3)-t15.*t94.*(2.1e+1./1.0e+3)+t94.*t252+t94.*t256+t94.*t259+t94.*t261+8.229e-1;
mt1 = [3.9e+1./5.0,0.0,0.0,t1427,t1421,t1425,t1267,t1385,t1394,0.0,0.0,0.0,t1268,t1386,t1395,0.0,0.0,0.0,t1269,t1387,t1396,0.0,0.0,0.0,t1270,t1388,t1397,0.0,0.0,0.0,0.0,3.9e+1./5.0,0.0,t1426,t1422,t1424,t1280,t1389,t1380,0.0,0.0,0.0,t1281,t1390,t1381,0.0,0.0,0.0,t1282,t1391,t1382,0.0,0.0,0.0,t1283,t1392,t1383,0.0,0.0,0.0,0.0,0.0,3.9e+1./5.0,0.0,t1423,t1409,t1133,t1332,t1341,0.0,0.0,0.0,t1134,t1333,t1342,0.0,0.0,0.0,t1135,t1334,t1343,0.0,0.0,0.0,t1136,t1335,t1344,0.0,0.0,0.0,t1427,t1426,0.0,et1+et2+et3+et4+et5+et6,t1430,t1429,t1384,t1400,t1404,0.0,0.0,0.0,t1398,t1401,t1405,0.0,0.0,0.0,t1399,t1402,t1406,0.0,0.0,0.0,t1393,t1403,t1407,0.0,0.0,0.0,t1421,t1422,t1423,t1430,et7+et8+et9+et10+et11+et12,t1428,t1345,t1410,t1412,0.0,0.0,0.0,t1336,t1413,t1416,0.0,0.0,0.0,t1346,t1417,t1414,0.0,0.0,0.0,t1347,t1415,t1411,0.0,0.0,0.0,t1425,t1424,t1409,t1429,t1428,et13+et14,t323,t1378,t1374,0.0,0.0,0.0,t254,t1376,t1368,0.0,0.0,0.0,t257,t1377,t1369,0.0,0.0,0.0,t326,t1379,t1375];
mt2 = [0.0,0.0,0.0,t1267,t1280,t1133,t1384,t1345,t323,4.0./3.75e+2,0.0,0.0,0.0,0.0,0.0,0.0,0.0,0.0,0.0,0.0,0.0,0.0,0.0,0.0,0.0,0.0,0.0,0.0,0.0,0.0,0.0,0.0,0.0,t1385,t1389,t1332,t1400,t1410,t1378,0.0,4.0./3.75e+2,0.0,0.0,0.0,0.0,0.0,0.0,0.0,0.0,0.0,0.0,0.0,0.0,0.0,0.0,0.0,0.0,0.0,0.0,0.0,0.0,0.0,0.0,t1394,t1380,t1341,t1404,t1412,t1374,0.0,0.0,4.0./3.75e+2,0.0,0.0,0.0,0.0,0.0,0.0,0.0,0.0,0.0,0.0,0.0,0.0,0.0,0.0,0.0,0.0,0.0,0.0,0.0,0.0,0.0,0.0,0.0,0.0,0.0,0.0,0.0,0.0,0.0,0.0,9.0./2.0e+1,0.0,0.0,0.0,0.0,0.0,0.0,0.0,0.0,0.0,0.0,0.0,0.0,0.0,0.0,0.0,0.0,0.0,0.0,0.0,0.0,0.0,0.0,0.0,0.0,0.0,0.0,0.0,0.0,0.0,0.0,9.0./2.0e+1,0.0,0.0,0.0,0.0,0.0,0.0,0.0,0.0,0.0,0.0,0.0,0.0,0.0,0.0,0.0,0.0,0.0,0.0,0.0,0.0,0.0,0.0,0.0,0.0,0.0,0.0,0.0,0.0,0.0,0.0,9.0./2.0e+1,0.0,0.0,0.0,0.0,0.0,0.0,0.0,0.0,0.0,0.0,0.0];
mt3 = [0.0,0.0,0.0,0.0,0.0,0.0,0.0,t1268,t1281,t1134,t1398,t1336,t254,0.0,0.0,0.0,0.0,0.0,0.0,4.0./3.75e+2,0.0,0.0,0.0,0.0,0.0,0.0,0.0,0.0,0.0,0.0,0.0,0.0,0.0,0.0,0.0,0.0,0.0,t1386,t1390,t1333,t1401,t1413,t1376,0.0,0.0,0.0,0.0,0.0,0.0,0.0,4.0./3.75e+2,0.0,0.0,0.0,0.0,0.0,0.0,0.0,0.0,0.0,0.0,0.0,0.0,0.0,0.0,0.0,0.0,t1395,t1381,t1342,t1405,t1416,t1368,0.0,0.0,0.0,0.0,0.0,0.0,0.0,0.0,4.0./3.75e+2,0.0,0.0,0.0,0.0,0.0,0.0,0.0,0.0,0.0,0.0,0.0,0.0,0.0,0.0,0.0,0.0,0.0,0.0,0.0,0.0,0.0,0.0,0.0,0.0,0.0,0.0,0.0,0.0,0.0,0.0,9.0./2.0e+1,0.0,0.0,0.0,0.0,0.0,0.0,0.0,0.0,0.0,0.0,0.0,0.0,0.0,0.0,0.0,0.0,0.0,0.0,0.0,0.0,0.0,0.0,0.0,0.0,0.0,0.0,0.0,0.0,0.0,0.0,9.0./2.0e+1,0.0,0.0,0.0,0.0,0.0,0.0,0.0,0.0,0.0,0.0,0.0,0.0,0.0,0.0,0.0,0.0,0.0,0.0,0.0,0.0,0.0,0.0,0.0,0.0,0.0,0.0,0.0,0.0,0.0,0.0,9.0./2.0e+1,0.0];
mt4 = [0.0,0.0,0.0,0.0,0.0,0.0,0.0,0.0,0.0,0.0,0.0,t1269,t1282,t1135,t1399,t1346,t257,0.0,0.0,0.0,0.0,0.0,0.0,0.0,0.0,0.0,0.0,0.0,0.0,4.0./3.75e+2,0.0,0.0,0.0,0.0,0.0,0.0,0.0,0.0,0.0,0.0,0.0,t1387,t1391,t1334,t1402,t1417,t1377,0.0,0.0,0.0,0.0,0.0,0.0,0.0,0.0,0.0,0.0,0.0,0.0,0.0,4.0./3.75e+2,0.0,0.0,0.0,0.0,0.0,0.0,0.0,0.0,0.0,0.0,t1396,t1382,t1343,t1406,t1414,t1369,0.0,0.0,0.0,0.0,0.0,0.0,0.0,0.0,0.0,0.0,0.0,0.0,0.0,0.0,4.0./3.75e+2,0.0,0.0,0.0,0.0,0.0,0.0,0.0,0.0,0.0,0.0,0.0,0.0,0.0,0.0,0.0,0.0,0.0,0.0,0.0,0.0,0.0,0.0,0.0,0.0,0.0,0.0,0.0,0.0,0.0,0.0,9.0./2.0e+1,0.0,0.0,0.0,0.0,0.0,0.0,0.0,0.0,0.0,0.0,0.0,0.0,0.0,0.0,0.0,0.0,0.0,0.0,0.0,0.0,0.0,0.0,0.0,0.0,0.0,0.0,0.0,0.0,0.0,0.0,9.0./2.0e+1,0.0,0.0,0.0,0.0,0.0,0.0,0.0,0.0,0.0,0.0,0.0,0.0,0.0,0.0,0.0,0.0,0.0,0.0,0.0,0.0,0.0,0.0,0.0,0.0,0.0,0.0];
mt5 = [0.0,0.0,0.0,0.0,9.0./2.0e+1,0.0,0.0,0.0,0.0,0.0,0.0,t1270,t1283,t1136,t1393,t1347,t326,0.0,0.0,0.0,0.0,0.0,0.0,0.0,0.0,0.0,0.0,0.0,0.0,0.0,0.0,0.0,0.0,0.0,0.0,4.0./3.75e+2,0.0,0.0,0.0,0.0,0.0,t1388,t1392,t1335,t1403,t1415,t1379,0.0,0.0,0.0,0.0,0.0,0.0,0.0,0.0,0.0,0.0,0.0,0.0,0.0,0.0,0.0,0.0,0.0,0.0,0.0,4.0./3.75e+2,0.0,0.0,0.0,0.0,t1397,t1383,t1344,t1407,t1411,t1375,0.0,0.0,0.0,0.0,0.0,0.0,0.0,0.0,0.0,0.0,0.0,0.0,0.0,0.0,0.0,0.0,0.0,0.0,0.0,0.0,4.0./3.75e+2,0.0,0.0,0.0,0.0,0.0,0.0,0.0,0.0,0.0,0.0,0.0,0.0,0.0,0.0,0.0,0.0,0.0,0.0,0.0,0.0,0.0,0.0,0.0,0.0,0.0,0.0,0.0,0.0,0.0,0.0,9.0./2.0e+1,0.0,0.0,0.0,0.0,0.0,0.0,0.0,0.0,0.0,0.0,0.0,0.0,0.0,0.0,0.0,0.0,0.0,0.0,0.0,0.0,0.0,0.0,0.0,0.0,0.0,0.0,0.0,0.0,0.0,0.0,9.0./2.0e+1,0.0,0.0,0.0,0.0,0.0,0.0,0.0,0.0,0.0,0.0,0.0,0.0,0.0,0.0,0.0,0.0];
mt6 = [0.0,0.0,0.0,0.0,0.0,0.0,0.0,0.0,0.0,0.0,0.0,0.0,0.0,0.0,9.0./2.0e+1];
M = reshape([mt1,mt2,mt3,mt4,mt5,mt6],30,30);
end
